simulink model "sim_dist_pos_obs_paper"  (R2020a)
settings: Solver=ode4  StartTime=0.0  StopTime=30.0  FixedStep=0.01  RelTol=1e-3
values from neighbouring files (symbols this model uses):
  alfa_theta = 20    [draw_compare_dist_pos_obs.m]
  alfa_theta_obs = 100    [draw_compare_dist_pos_obs.m]
  beta1 = 1.2    [draw_compare_dist_pos_obs.m]
  beta2 = 0.8    [draw_compare_dist_pos_obs.m]
  c1_diff_sigma_bar_v = diag([25; 30; 20])    [draw_compare_dist_pos_obs.m]
  c1v = diag([16.0; 16.0; 16.0])    [draw_compare_dist_pos_obs.m]
  c2_diff_sigma_bar_v = diag([50; 50; 10])    [draw_compare_dist_pos_obs.m]
  c2v = diag([16.0; 16.0; 16.0])    [draw_compare_dist_pos_obs.m]
  c3_diff_sigma_bar_v = diag([15; 15; 10])    [draw_compare_dist_pos_obs.m]
  c3v = diag([16.0; 16.0; 16.0])    [draw_compare_dist_pos_obs.m]
  delta_p_i_0 = zeros(3, NF)    [draw_compare_dist_pos_obs.m]
  delta_v_i_0 = zeros(3, NF)    [draw_compare_dist_pos_obs.m]
  dp_aa_t = 0.2 * ones(3, 5) + ( 1.0 - 0.2 ) * rand(3, 5)    [draw_compare_dist_pos_obs.m]
  dp_ff_t = [ 0.4 * ones(1, 5) + ( 1.0 - 0.4 ) * rand(1, 5);                      0.4 * ones(1, 5) + ( 1.0 - 0.4 ) * rand(1, 5);                      0.2 * ones(1, 5) + ( 0.6 - 0.2 ) * rand(1, 5) ]    [draw_compare_dist_pos_obs.m]
  dp_phi_t = ( - pi / 2 ) * ones(3, 5) + ( pi / 2 - ( - pi / 2 ) ) * rand(3, 5)    [draw_compare_dist_pos_obs.m]
  etai_0 = zeros(3,5)    [draw_compare_dist_pos_obs.m]
  kai_1_t = 0.02    [draw_compare_dist_pos_obs.m]
  kai_3_t = 0.1    [draw_compare_dist_pos_obs.m]
  kai_chi_1 = diag([6; 6; 6])    [draw_compare_dist_pos_obs.m]
  kai_chi_2 = diag([6; 6; 6])    [draw_compare_dist_pos_obs.m]
  kai_u_1 = diag([8; 8; 8])    [draw_compare_dist_pos_obs.m]
  kai_u_2 = diag([8; 8; 8])    [draw_compare_dist_pos_obs.m]
  ksii_0 = zeros(3,5)    [draw_compare_dist_pos_obs.m]
  l1v = diag([20; 20; 20])    [draw_compare_dist_pos_obs.m]
  l2v = diag([30; 30; 30])    [draw_compare_dist_pos_obs.m]
  Lamd_diff_sigma_bar_v = 0.5    [draw_compare_dist_pos_obs.m]
  mass_i = zeros(1,NF)    [draw_compare_dist_pos_obs.m]
  Mii = diag([1;0;0;0;1])    [draw_compare_dist_pos_obs.m]
  pos0 = zeros(3, 1)    [draw_compare_dist_pos_obs.m]
  PZ0 = P0(3)    [draw_compare_dist_pos_obs.m]
  PZ1 = 10    [draw_compare_dist_pos_obs.m]
  Qci_init = repmat([1;0;0;0],1,NF)    [draw_compare_dist_pos_obs.m]
  R0 = 4    [draw_compare_dist_pos_obs.m]
  R1 = 8    [draw_compare_dist_pos_obs.m]
  Rx2 = 10    [draw_compare_dist_pos_obs.m]
  Ry2 = 6    [draw_compare_dist_pos_obs.m]
  Rz2 = 4    [draw_compare_dist_pos_obs.m]
  T0 = 0    [draw_compare_dist_pos_obs.m]
  T1 = tseq1    (= 10)    [draw_compare_dist_pos_obs.m]
  T12 = tseq1 + tseq12    (= 20)    [draw_compare_dist_pos_obs.m]
  T2 = tseq1 + tseq12 + tseq2    (= 30)    [draw_compare_dist_pos_obs.m]
  theta0 = ( 2 / 5 ) * pi    (= 1.25663706144)    [draw_compare_dist_pos_obs.m]
  vel0 = zeros(3, 1)    [draw_compare_dist_pos_obs.m]
  Wij = [0,0,1,0,0;              0,0,1,1,0;              1,0,0,0,1;              0,1,1,0,0;              0,0,1,0,0]    [draw_compare_dist_pos_obs.m]
  X1 = 8    [draw_compare_dist_pos_obs.m]
  X2 = 2    [draw_compare_dist_pos_obs.m]
  X3 = 3    [draw_compare_dist_pos_obs.m]
  Y1 = 10    [draw_compare_dist_pos_obs.m]
  Y2 = 2    [draw_compare_dist_pos_obs.m]
  Y3 = 4    [draw_compare_dist_pos_obs.m]
  Z1 = 4    [draw_compare_dist_pos_obs.m]
  Z2 = -6    [draw_compare_dist_pos_obs.m]
  Z3 = 2    [draw_compare_dist_pos_obs.m]
  zeta_diff_sigma_bar_v = 0.08    [draw_compare_dist_pos_obs.m]
undefined symbols (not defined in the file or in its folder): cal_frac_squ, p_alfav1, p_alfav2, p_beta1, p_beta2, p_dbeta1, p_dbeta2, p_gamma1_pos, p_gamma1_vel, p_gamma2_pos, p_gamma2_vel, q_alfav1, q_alfav2, q_beta1, q_beta2, q_dbeta1, q_dbeta2, q_gamma1_pos, q_gamma1_vel, q_gamma2_pos, q_gamma2_vel
(part 1 of 5)
settings Model: Creator=zzy  LastModifiedBy=Hershey.A
settings DataIOCC: ReturnWorkspaceOutputs=off
settings DebuggingCC: ArithmeticOperatorsInVariantConditions=warning
settings SFSimCC: SimUseLocalCustomCode=off  CustomCodeUndefinedFunction=UseInterfaceOnly
settings RTWCC: RTWUseLocalCustomCode=off

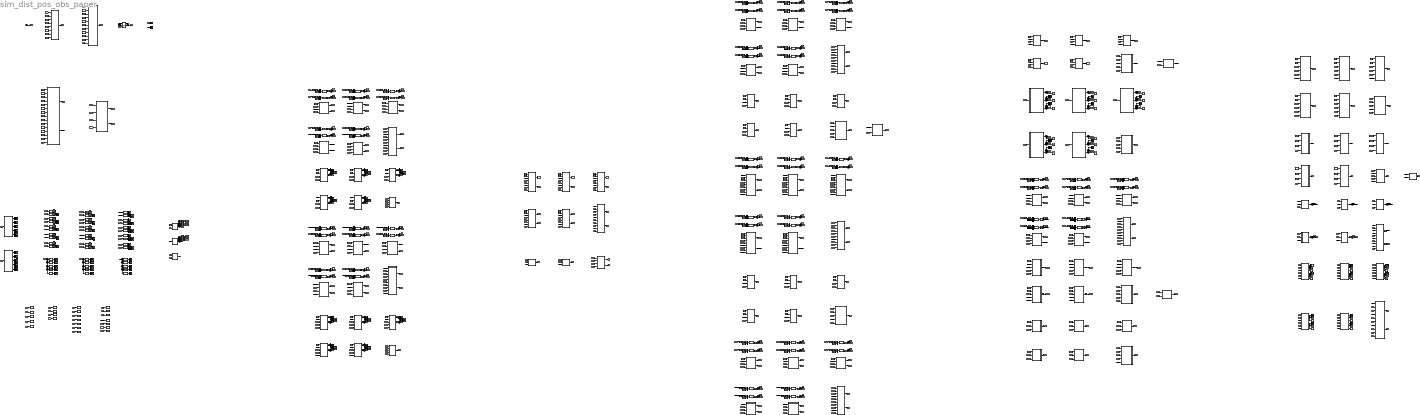
== system sim_dist_pos_obs_paper ==
  Add{,1..9} (10 alike) : Sum
  Clock : Clock
  Constant : Constant  Value=T1
  Constant{1,4,9,19,24,149,154,159,164,169} (10 alike) : Constant  Value=q_beta1
  Constant{5,10,14,16,20,39,46,54,61,79,101,103,108,113,118,148,153,158,163,168} (20 alike) : Constant  Value=alfa_theta
  Constant{100,102,107,112,117} (5 alike) : Constant  Value=p_alfav1
  Constant{97,104,109,114,119} (5 alike) : Constant  Value=q_alfav1
  Constant{98,105,110,115,120} (5 alike) : Constant  Value=p_alfav2
  Constant{99,106,111,116,121} (5 alike) : Constant  Value=q_alfav2
  Constant{2,6,11,15,21,150,155,160,165,170} (10 alike) : Constant  Value=p_beta2
  Constant{3,7,12,17,22,151,156,161,166,171} (10 alike) : Constant  Value=q_beta2
  Constant{122,124,126,128,140} (5 alike) : Constant  Value=c1v
  Constant{123,125,127,139,141} (5 alike) : Constant  Value=c2v
  Constant129 : Constant  Value=R0
  Constant{8,13,18,23,63,147,152,157,162,167} (10 alike) : Constant  Value=p_beta1
  Constant130 : Constant  Value=R1
  Constant131 : Constant  Value=T0
  Constant132 : Constant  Value=Rz2
  Constant133 : Constant  Value=Ry2
  Constant134 : Constant  Value=Rx2
  Constant135 : Constant  Value=X1
  Constant136 : Constant  Value=X2
  Constant137 : Constant  Value=Y1
  Constant138 : Constant  Value=Y2
  Constant{92..96,142..146} (10 alike) : Constant  Value=c3v
  Constant{172,174,176,178,180} (5 alike) : Constant  Value=kai_u_1
  Constant{173,175,177,179,181} (5 alike) : Constant  Value=kai_u_2
  Constant{182..183,189,199,202,205,209,212,219,252} (10 alike) : Constant  Value=l2v
  Constant{184..186,193..196,198,283..284} (10 alike) : Constant  Value=alfa_theta_obs
  Constant{187,190,197,200,203,206,210,213,230,263} (10 alike) : Constant  Value=l1v
  Constant188 : Constant  Value=delta_p_i_0(:,4)
  Constant191 : Constant  Value=mass_i
  Constant192 : Constant  Value=delta_p_i_0(:,5)
  Constant201 : Constant  Value=delta_v_i_0(:,1)
  Constant204 : Constant  Value=delta_v_i_0(:,2)
  Constant207 : Constant  Value=delta_v_i_0(:,3)
  Constant208 : Constant  Value=delta_p_i_0(:,1)
  Constant211 : Constant  Value=delta_v_i_0(:,4)
  Constant214 : Constant  Value=delta_v_i_0(:,5)
  Constant{215,220,270,275,279} (5 alike) : Constant  Value=p_gamma1_pos
  Constant{216,267,271,276,280} (5 alike) : Constant  Value=q_gamma1_pos
  Constant{217,268,272,277,281} (5 alike) : Constant  Value=p_gamma2_pos
  Constant{218,269,273,278,282} (5 alike) : Constant  Value=q_gamma2_pos
  Constant221 : Constant  Value=Z1
  Constant222 : Constant  Value=Z2
  Constant{223,227,232,236,240} (5 alike) : Constant  Value=Wij
  Constant{224,228,233,237,242} (5 alike) : Constant  Value=Mii
  Constant225 : Constant  Value=theta0
  Constant226 : Constant  Value=Z3
  Constant229 : Constant  Value=Y3
  Constant231 : Constant  Value=kai_1_t
  Constant234 : Constant  Value=X3
  Constant235 : Constant  Value=kai_3_t
  Constant238 : Constant  Value=T1
  Constant239 : Constant  Value=T12
  Constant241 : Constant  Value=delta_p_i_0(:,2)
  Constant{243,286,289,292,295} (5 alike) : Constant  Value=dp_phi_t
  Constant{244,287,290,293,296} (5 alike) : Constant  Value=dp_ff_t
  Constant{245,249,254,258,262} (5 alike) : Constant  Value=p_gamma1_vel
  Constant{246,250,255,259,264} (5 alike) : Constant  Value=q_gamma1_vel
  Constant{247,251,256,260,265} (5 alike) : Constant  Value=p_gamma2_vel
  Constant{248,253,257,261,266} (5 alike) : Constant  Value=q_gamma2_vel
  Constant{25,27,29,31,33,82,84,86,88,90} (10 alike) : Constant  Value=kai_chi_2
  Constant{26,28,30,32,34,83,85,87,89,91} (10 alike) : Constant  Value=kai_chi_1
  Constant274 : Constant  Value=delta_p_i_0(:,3)
  Constant{285,288,291,294,297} (5 alike) : Constant  Value=dp_aa_t
  Constant{35,42,49,57,75} (5 alike) : Constant  Value=q_dbeta1
  Constant{36,43,50,58,76} (5 alike) : Constant  Value=p_dbeta2
  Constant{37,44,52,59,77} (5 alike) : Constant  Value=q_dbeta2
  Constant{38,45,53,60,78} (5 alike) : Constant  Value=p_dbeta1
  Constant{40,47,55,62,80} (5 alike) : Constant  Value=beta1
  Constant{41,48,56,74,81} (5 alike) : Constant  Value=beta2
  Constant51 : Constant  Value=Qci_init
  Constant64 : Constant  Value=T2
  Constant65 : Constant  Value=R0
  Constant66 : Constant  Value=R1
  Constant67 : Constant  Value=Rx2
  Constant68 : Constant  Value=Ry2
  Constant69 : Constant  Value=Rz2
  Constant70 : Constant  Value=T2
  Constant71 : Constant  Value=T1
  Constant72 : Constant  Value=PZ0
  Constant73 : Constant  Value=PZ1
  Demux{1..97} (97 alike) : Demux  Outputs=3
  Display{1..95} (95 alike) : Display
  Interpreted MATLAB Function{1..60} (60 alike) : MATLABFcn  MATLABFcn=cal_frac_squ(u(1:3),u(4),u(5))
  Memory1 : Memory  InitialCondition=etai_0
  Memory2 : Memory  InitialCondition=ksii_0
  Mux{1..40,109..118,120..129} (60 alike) : Mux  Inputs=3
  Mux{41..108,119,130..135} (75 alike) : Mux  Inputs=2
  Step : Step  Time=T1+0.01  SampleTime=0
  To Workspace : ToWorkspace  VariableName=eta_d_est_vec  SampleTime=-1
  To Workspace1 : ToWorkspace  VariableName=dp_hat_vec  SampleTime=-1
  To Workspace10 : ToWorkspace  VariableName=eta_track_err_vec  SampleTime=-1
  To Workspace11 : ToWorkspace  VariableName=sigma_bar_v_hat_vec  SampleTime=-1
  To Workspace12 : ToWorkspace  VariableName=sigma_bar_v_vec  SampleTime=-1
  To Workspace13 : ToWorkspace  VariableName=sigma_bar_v_tilt_vec  SampleTime=-1
  To Workspace14 : ToWorkspace  VariableName=ui_vec  SampleTime=-1
  To Workspace15 : ToWorkspace  VariableName=chi_vec  SampleTime=-1
  To Workspace16 : ToWorkspace  VariableName=phi_vec  SampleTime=-1
  To Workspace17 : ToWorkspace  VariableName=ksi_est_err  SampleTime=-1
  To Workspace18 : ToWorkspace  VariableName=ksi_d_est_vec  SampleTime=-1
  To Workspace19 : ToWorkspace  VariableName=sigma_v_vec  SampleTime=-1
  To Workspace2 : ToWorkspace  VariableName=dp_vec  SampleTime=-1
  To Workspace20 : ToWorkspace  VariableName=delta_ksi_vec  SampleTime=-1
  To Workspace21 : ToWorkspace  VariableName=delta_eta_vec  SampleTime=-1
  To Workspace22 : ToWorkspace  VariableName=eta_est_err  SampleTime=-1
  To Workspace3 : ToWorkspace  VariableName=u0  SampleTime=-1
  To Workspace4 : ToWorkspace  VariableName=eta0  SampleTime=-1
  To Workspace5 : ToWorkspace  VariableName=ksi0  SampleTime=-1
  To Workspace6 : ToWorkspace  VariableName=dp_tilt_vec  SampleTime=-1
  To Workspace7 : ToWorkspace  VariableName=eta_i_vec  SampleTime=-1
  To Workspace8 : ToWorkspace  VariableName=ksi_i_vec  SampleTime=-1
  To Workspace9 : ToWorkspace  VariableName=ksi_track_err_vec  SampleTime=-1
  cal Rci from ui : MATLAB Function  TreatAsAtomicUnit=on
  cal Rei : MATLAB Function  TreatAsAtomicUnit=on
  cal Ri : MATLAB Function  TreatAsAtomicUnit=on
  cal abs 1 : MATLAB Function  TreatAsAtomicUnit=on
  cal abs 10 : MATLAB Function  TreatAsAtomicUnit=on
  cal abs 11 : MATLAB Function  TreatAsAtomicUnit=on
  cal abs 12 : MATLAB Function  TreatAsAtomicUnit=on
  cal abs 13 : MATLAB Function  TreatAsAtomicUnit=on
  cal abs 14 : MATLAB Function  TreatAsAtomicUnit=on
  cal abs 15 : MATLAB Function  TreatAsAtomicUnit=on
  cal abs 16 : MATLAB Function  TreatAsAtomicUnit=on
  cal abs 17 : MATLAB Function  TreatAsAtomicUnit=on
  cal abs 18 : MATLAB Function  TreatAsAtomicUnit=on
  cal abs 19 : MATLAB Function  TreatAsAtomicUnit=on
  cal abs 2 : MATLAB Function  TreatAsAtomicUnit=on
  cal abs 20 : MATLAB Function  TreatAsAtomicUnit=on
  cal abs 21 : MATLAB Function  TreatAsAtomicUnit=on
  cal abs 22 : MATLAB Function  TreatAsAtomicUnit=on
  cal abs 23 : MATLAB Function  TreatAsAtomicUnit=on
  cal abs 24 : MATLAB Function  TreatAsAtomicUnit=on
  cal abs 25 : MATLAB Function  TreatAsAtomicUnit=on
  cal abs 26 : MATLAB Function  TreatAsAtomicUnit=on
  cal abs 27 : MATLAB Function  TreatAsAtomicUnit=on
  cal abs 28 : MATLAB Function  TreatAsAtomicUnit=on
  cal abs 29 : MATLAB Function  TreatAsAtomicUnit=on
  cal abs 3 : MATLAB Function  TreatAsAtomicUnit=on
  cal abs 30 : MATLAB Function  TreatAsAtomicUnit=on
  cal abs 31 : MATLAB Function  TreatAsAtomicUnit=on
  cal abs 32 : MATLAB Function  TreatAsAtomicUnit=on
  cal abs 33 : MATLAB Function  TreatAsAtomicUnit=on
  cal abs 34 : MATLAB Function  TreatAsAtomicUnit=on
  cal abs 35 : MATLAB Function  TreatAsAtomicUnit=on
  cal abs 36 : MATLAB Function  TreatAsAtomicUnit=on
  cal abs 37 : MATLAB Function  TreatAsAtomicUnit=on
  cal abs 38 : MATLAB Function  TreatAsAtomicUnit=on
  cal abs 39 : MATLAB Function  TreatAsAtomicUnit=on
  cal abs 4 : MATLAB Function  TreatAsAtomicUnit=on
  cal abs 40 : MATLAB Function  TreatAsAtomicUnit=on
  cal abs 41 : MATLAB Function  TreatAsAtomicUnit=on
  cal abs 42 : MATLAB Function  TreatAsAtomicUnit=on
  cal abs 43 : MATLAB Function  TreatAsAtomicUnit=on
  cal abs 44 : MATLAB Function  TreatAsAtomicUnit=on
  cal abs 45 : MATLAB Function  TreatAsAtomicUnit=on
  cal abs 46 : MATLAB Function  TreatAsAtomicUnit=on
  cal abs 47 : MATLAB Function  TreatAsAtomicUnit=on
  cal abs 48 : MATLAB Function  TreatAsAtomicUnit=on
  cal abs 49 : MATLAB Function  TreatAsAtomicUnit=on
  cal abs 5 : MATLAB Function  TreatAsAtomicUnit=on
  cal abs 50 : MATLAB Function  TreatAsAtomicUnit=on
  cal abs 51 : MATLAB Function  TreatAsAtomicUnit=on
  cal abs 52 : MATLAB Function  TreatAsAtomicUnit=on
  cal abs 53 : MATLAB Function  TreatAsAtomicUnit=on
  cal abs 54 : MATLAB Function  TreatAsAtomicUnit=on
  cal abs 55 : MATLAB Function  TreatAsAtomicUnit=on
  cal abs 56 : MATLAB Function  TreatAsAtomicUnit=on
  cal abs 57 : MATLAB Function  TreatAsAtomicUnit=on
  cal abs 58 : MATLAB Function  TreatAsAtomicUnit=on
  cal abs 59 : MATLAB Function  TreatAsAtomicUnit=on
  cal abs 6 : MATLAB Function  TreatAsAtomicUnit=on
  cal abs 60 : MATLAB Function  TreatAsAtomicUnit=on
  cal abs 7 : MATLAB Function  TreatAsAtomicUnit=on
  cal abs 8 : MATLAB Function  TreatAsAtomicUnit=on
  cal abs 9 : MATLAB Function  TreatAsAtomicUnit=on
  cal combine sigma_bar_v : MATLAB Function  TreatAsAtomicUnit=on
  cal combine sigma_bar_v_tilt : MATLAB Function  TreatAsAtomicUnit=on
  cal d_theta_err_ksi agent 1 : MATLAB Function  TreatAsAtomicUnit=on
  cal d_theta_err_ksi agent 2 : MATLAB Function  TreatAsAtomicUnit=on
  cal d_theta_err_ksi agent 3 : MATLAB Function  TreatAsAtomicUnit=on
  cal d_theta_err_ksi agent 4 : MATLAB Function  TreatAsAtomicUnit=on
  cal d_theta_err_ksi agent 5 : MATLAB Function  TreatAsAtomicUnit=on
  cal dchi agent 1 : MATLAB Function  TreatAsAtomicUnit=on
  cal dchi agent 2 : MATLAB Function  TreatAsAtomicUnit=on
  cal dchi agent 3 : MATLAB Function  TreatAsAtomicUnit=on
  cal dchi agent 4 : MATLAB Function  TreatAsAtomicUnit=on
  cal dchi agent 5 : MATLAB Function  TreatAsAtomicUnit=on
  cal differentiator d_sigma_bar_v_hat agent 1 : Subsystem
  cal differentiator d_sigma_bar_v_hat agent 2 : Subsystem
  cal differentiator d_sigma_bar_v_hat agent 3 : Subsystem
  cal differentiator d_sigma_bar_v_hat agent 4 : Subsystem
  cal differentiator d_sigma_bar_v_hat agent 5 : Subsystem
  cal disturbance observation error dp_tilt : MATLAB Function  TreatAsAtomicUnit=on
  cal dp_hat agent 1 : MATLAB Function  TreatAsAtomicUnit=on
  cal dp_hat agent 2 : MATLAB Function  TreatAsAtomicUnit=on
  cal dp_hat agent 3 : MATLAB Function  TreatAsAtomicUnit=on
  cal dp_hat agent 4 : MATLAB Function  TreatAsAtomicUnit=on
  cal dp_hat agent 5 : MATLAB Function  TreatAsAtomicUnit=on
  cal formation tracking position and velocity errors : MATLAB Function  TreatAsAtomicUnit=on
  cal lumped observation error agent 1 : MATLAB Function  TreatAsAtomicUnit=on
  cal lumped observation error agent 2 : MATLAB Function  TreatAsAtomicUnit=on
  cal lumped observation error agent 3 : MATLAB Function  TreatAsAtomicUnit=on
  cal lumped observation error agent 4 : MATLAB Function  TreatAsAtomicUnit=on
  cal lumped observation error agent 5 : MATLAB Function  TreatAsAtomicUnit=on
  cal position estimate error : MATLAB Function  TreatAsAtomicUnit=on
  cal sigma_bar_v_hat agent 1 : MATLAB Function  TreatAsAtomicUnit=on
  cal sigma_bar_v_hat agent 2 : MATLAB Function  TreatAsAtomicUnit=on
  cal sigma_bar_v_hat agent 3 : MATLAB Function  TreatAsAtomicUnit=on
  cal sigma_bar_v_hat agent 4 : MATLAB Function  TreatAsAtomicUnit=on
  cal sigma_bar_v_hat agent 5 : MATLAB Function  TreatAsAtomicUnit=on
  cal theta_err_ksi agent 1 : MATLAB Function  TreatAsAtomicUnit=on
  cal theta_err_ksi agent 2 : MATLAB Function  TreatAsAtomicUnit=on
  cal theta_err_ksi agent 3 : MATLAB Function  TreatAsAtomicUnit=on
  cal theta_err_ksi agent 4 : MATLAB Function  TreatAsAtomicUnit=on
  cal theta_err_ksi agent 5 : MATLAB Function  TreatAsAtomicUnit=on
  cal theta_eta_est_err_tilt agent 1 : MATLAB Function  TreatAsAtomicUnit=on
  cal theta_eta_est_err_tilt agent 2 : MATLAB Function  TreatAsAtomicUnit=on
  cal theta_eta_est_err_tilt agent 3 : MATLAB Function  TreatAsAtomicUnit=on
  cal theta_eta_est_err_tilt agent 4 : MATLAB Function  TreatAsAtomicUnit=on
  cal theta_eta_est_err_tilt agent 5 : MATLAB Function  TreatAsAtomicUnit=on
  cal theta_ksi_est_err_tilt agent 1 : MATLAB Function  TreatAsAtomicUnit=on
  cal theta_ksi_est_err_tilt agent 2 : MATLAB Function  TreatAsAtomicUnit=on
  cal theta_ksi_est_err_tilt agent 3 : MATLAB Function  TreatAsAtomicUnit=on
  cal theta_ksi_est_err_tilt agent 4 : MATLAB Function  TreatAsAtomicUnit=on
  cal theta_ksi_est_err_tilt agent 5 : MATLAB Function  TreatAsAtomicUnit=on
  cal theta_phi agent 1 : MATLAB Function  TreatAsAtomicUnit=on
  cal theta_phi agent 2 : MATLAB Function  TreatAsAtomicUnit=on
  cal theta_phi agent 3 : MATLAB Function  TreatAsAtomicUnit=on
  cal theta_phi agent 4 : MATLAB Function  TreatAsAtomicUnit=on
  cal theta_phi agent 5 : MATLAB Function  TreatAsAtomicUnit=on
  cal theta_sigma_bar_v_tilt agent 1 : MATLAB Function  TreatAsAtomicUnit=on
  cal theta_sigma_bar_v_tilt agent 2 : MATLAB Function  TreatAsAtomicUnit=on
  cal theta_sigma_bar_v_tilt agent 3 : MATLAB Function  TreatAsAtomicUnit=on
  cal theta_sigma_bar_v_tilt agent 4 : MATLAB Function  TreatAsAtomicUnit=on
  cal theta_sigma_bar_v_tilt agent 5 : MATLAB Function  TreatAsAtomicUnit=on
  cal ui agent 1 : MATLAB Function  TreatAsAtomicUnit=on
  cal ui agent 2 : MATLAB Function  TreatAsAtomicUnit=on
  cal ui agent 3 : MATLAB Function  TreatAsAtomicUnit=on
  cal ui agent 4 : MATLAB Function  TreatAsAtomicUnit=on
  cal ui agent 5 : MATLAB Function  TreatAsAtomicUnit=on
  cal velocity estimate error : MATLAB Function  TreatAsAtomicUnit=on
  cal virtual control sigma_v agent 1 : MATLAB Function  TreatAsAtomicUnit=on
  cal virtual control sigma_v agent 2 : MATLAB Function  TreatAsAtomicUnit=on
  cal virtual control sigma_v agent 3 : MATLAB Function  TreatAsAtomicUnit=on
  cal virtual control sigma_v agent 4 : MATLAB Function  TreatAsAtomicUnit=on
  cal virtual control sigma_v agent 5 : MATLAB Function  TreatAsAtomicUnit=on
  cal virtual velocity control error phi : MATLAB Function  TreatAsAtomicUnit=on
  choose chi_1 : MATLAB Function  TreatAsAtomicUnit=on
  choose chi_2 : MATLAB Function  TreatAsAtomicUnit=on
  choose chi_3 : MATLAB Function  TreatAsAtomicUnit=on
  choose chi_4 : MATLAB Function  TreatAsAtomicUnit=on
  choose chi_5 : MATLAB Function  TreatAsAtomicUnit=on
  choose dp_1 : MATLAB Function  TreatAsAtomicUnit=on
  choose dp_2 : MATLAB Function  TreatAsAtomicUnit=on
  choose dp_3 : MATLAB Function  TreatAsAtomicUnit=on
  choose dp_4 : MATLAB Function  TreatAsAtomicUnit=on
  choose dp_5 : MATLAB Function  TreatAsAtomicUnit=on
  choose dp_hat_1 : MATLAB Function  TreatAsAtomicUnit=on
  choose dp_hat_2 : MATLAB Function  TreatAsAtomicUnit=on
  choose dp_hat_3 : MATLAB Function  TreatAsAtomicUnit=on
  choose dp_hat_4 : MATLAB Function  TreatAsAtomicUnit=on
  choose dp_hat_5 : MATLAB Function  TreatAsAtomicUnit=on
  choose dp_tilt_1 : MATLAB Function  TreatAsAtomicUnit=on
  choose dp_tilt_2 : MATLAB Function  TreatAsAtomicUnit=on
  choose dp_tilt_3 : MATLAB Function  TreatAsAtomicUnit=on
  choose dp_tilt_4 : MATLAB Function  TreatAsAtomicUnit=on
  choose dp_tilt_5 : MATLAB Function  TreatAsAtomicUnit=on
  choose err_eta_1 : MATLAB Function  TreatAsAtomicUnit=on
  choose err_eta_2 : MATLAB Function  TreatAsAtomicUnit=on
  choose err_eta_3 : MATLAB Function  TreatAsAtomicUnit=on
  choose err_eta_4 : MATLAB Function  TreatAsAtomicUnit=on
  choose err_eta_5 : MATLAB Function  TreatAsAtomicUnit=on
  choose eta_est_err_tilt 1 : MATLAB Function  TreatAsAtomicUnit=on
  choose eta_est_err_tilt 10 : MATLAB Function  TreatAsAtomicUnit=on
  choose eta_est_err_tilt 11 : MATLAB Function  TreatAsAtomicUnit=on
  choose eta_est_err_tilt 12 : MATLAB Function  TreatAsAtomicUnit=on
  choose eta_est_err_tilt 13 : MATLAB Function  TreatAsAtomicUnit=on
  choose eta_est_err_tilt 14 : MATLAB Function  TreatAsAtomicUnit=on
  choose eta_est_err_tilt 15 : MATLAB Function  TreatAsAtomicUnit=on
  choose eta_est_err_tilt 16 : MATLAB Function  TreatAsAtomicUnit=on
  choose eta_est_err_tilt 17 : MATLAB Function  TreatAsAtomicUnit=on
  choose eta_est_err_tilt 18 : MATLAB Function  TreatAsAtomicUnit=on
  choose eta_est_err_tilt 19 : MATLAB Function  TreatAsAtomicUnit=on
  choose eta_est_err_tilt 2 : MATLAB Function  TreatAsAtomicUnit=on
  choose eta_est_err_tilt 20 : MATLAB Function  TreatAsAtomicUnit=on
  choose eta_est_err_tilt 3 : MATLAB Function  TreatAsAtomicUnit=on
  choose eta_est_err_tilt 4 : MATLAB Function  TreatAsAtomicUnit=on
  choose eta_est_err_tilt 5 : MATLAB Function  TreatAsAtomicUnit=on
  choose eta_est_err_tilt 6 : MATLAB Function  TreatAsAtomicUnit=on
  choose eta_est_err_tilt 7 : MATLAB Function  TreatAsAtomicUnit=on
  choose eta_est_err_tilt 8 : MATLAB Function  TreatAsAtomicUnit=on
  choose eta_est_err_tilt 9 : MATLAB Function  TreatAsAtomicUnit=on
  choose ksi_est_err 1 : MATLAB Function  TreatAsAtomicUnit=on
  choose ksi_est_err 10 : MATLAB Function  TreatAsAtomicUnit=on
  choose ksi_est_err 11 : MATLAB Function  TreatAsAtomicUnit=on
  choose ksi_est_err 12 : MATLAB Function  TreatAsAtomicUnit=on
  choose ksi_est_err 13 : MATLAB Function  TreatAsAtomicUnit=on
  choose ksi_est_err 14 : MATLAB Function  TreatAsAtomicUnit=on
  choose ksi_est_err 15 : MATLAB Function  TreatAsAtomicUnit=on
  choose ksi_est_err 16 : MATLAB Function  TreatAsAtomicUnit=on
  choose ksi_est_err 17 : MATLAB Function  TreatAsAtomicUnit=on
  choose ksi_est_err 18 : MATLAB Function  TreatAsAtomicUnit=on
  choose ksi_est_err 19 : MATLAB Function  TreatAsAtomicUnit=on
  choose ksi_est_err 2 : MATLAB Function  TreatAsAtomicUnit=on
  choose ksi_est_err 20 : MATLAB Function  TreatAsAtomicUnit=on
  choose ksi_est_err 21 : MATLAB Function  TreatAsAtomicUnit=on
  choose ksi_est_err 22 : MATLAB Function  TreatAsAtomicUnit=on
  choose ksi_est_err 23 : MATLAB Function  TreatAsAtomicUnit=on
  choose ksi_est_err 24 : MATLAB Function  TreatAsAtomicUnit=on
  choose ksi_est_err 25 : MATLAB Function  TreatAsAtomicUnit=on
  choose ksi_est_err 26 : MATLAB Function  TreatAsAtomicUnit=on
  choose ksi_est_err 27 : MATLAB Function  TreatAsAtomicUnit=on
  choose ksi_est_err 28 : MATLAB Function  TreatAsAtomicUnit=on
  choose ksi_est_err 29 : MATLAB Function  TreatAsAtomicUnit=on
  choose ksi_est_err 3 : MATLAB Function  TreatAsAtomicUnit=on
  choose ksi_est_err 30 : MATLAB Function  TreatAsAtomicUnit=on
  choose ksi_est_err 31 : MATLAB Function  TreatAsAtomicUnit=on
  choose ksi_est_err 32 : MATLAB Function  TreatAsAtomicUnit=on
  choose ksi_est_err 33 : MATLAB Function  TreatAsAtomicUnit=on
  choose ksi_est_err 34 : MATLAB Function  TreatAsAtomicUnit=on
  choose ksi_est_err 35 : MATLAB Function  TreatAsAtomicUnit=on
  choose ksi_est_err 36 : MATLAB Function  TreatAsAtomicUnit=on
  choose ksi_est_err 37 : MATLAB Function  TreatAsAtomicUnit=on
  choose ksi_est_err 38 : MATLAB Function  TreatAsAtomicUnit=on
  choose ksi_est_err 39 : MATLAB Function  TreatAsAtomicUnit=on
  choose ksi_est_err 4 : MATLAB Function  TreatAsAtomicUnit=on
  choose ksi_est_err 40 : MATLAB Function  TreatAsAtomicUnit=on
  choose ksi_est_err 5 : MATLAB Function  TreatAsAtomicUnit=on
  choose ksi_est_err 6 : MATLAB Function  TreatAsAtomicUnit=on
  choose ksi_est_err 7 : MATLAB Function  TreatAsAtomicUnit=on
  choose ksi_est_err 8 : MATLAB Function  TreatAsAtomicUnit=on
  choose ksi_est_err 9 : MATLAB Function  TreatAsAtomicUnit=on
  choose phi_1 : MATLAB Function  TreatAsAtomicUnit=on
  choose phi_2 : MATLAB Function  TreatAsAtomicUnit=on
  choose phi_3 : MATLAB Function  TreatAsAtomicUnit=on
  choose phi_4 : MATLAB Function  TreatAsAtomicUnit=on
  choose phi_5 : MATLAB Function  TreatAsAtomicUnit=on
  choose sigma_bar_v_1 : MATLAB Function  TreatAsAtomicUnit=on
  choose sigma_bar_v_2 : MATLAB Function  TreatAsAtomicUnit=on
  choose sigma_bar_v_3 : MATLAB Function  TreatAsAtomicUnit=on
  choose sigma_bar_v_4 : MATLAB Function  TreatAsAtomicUnit=on
  choose sigma_bar_v_5 : MATLAB Function  TreatAsAtomicUnit=on
  choose sigma_bar_v_hat_1 : MATLAB Function  TreatAsAtomicUnit=on
  choose sigma_bar_v_hat_2 : MATLAB Function  TreatAsAtomicUnit=on
  choose sigma_bar_v_hat_3 : MATLAB Function  TreatAsAtomicUnit=on
  choose sigma_bar_v_hat_4 : MATLAB Function  TreatAsAtomicUnit=on
  choose sigma_bar_v_hat_5 : MATLAB Function  TreatAsAtomicUnit=on
  choose sigma_bar_v_tilt_1 : MATLAB Function  TreatAsAtomicUnit=on
  choose sigma_bar_v_tilt_2 : MATLAB Function  TreatAsAtomicUnit=on
  choose sigma_bar_v_tilt_3 : MATLAB Function  TreatAsAtomicUnit=on
  choose sigma_bar_v_tilt_4 : MATLAB Function  TreatAsAtomicUnit=on
  choose sigma_bar_v_tilt_5 : MATLAB Function  TreatAsAtomicUnit=on
  combine chi : MATLAB Function  TreatAsAtomicUnit=on
  combine d_sigma_bar_v_est : MATLAB Function  TreatAsAtomicUnit=on
  combine dchi : MATLAB Function  TreatAsAtomicUnit=on
  combine dp_hat : MATLAB Function  TreatAsAtomicUnit=on
  combine dtheta_err_ksi : MATLAB Function  TreatAsAtomicUnit=on
  combine follower desire velocity estimaters : MATLAB Function  TreatAsAtomicUnit=on
  combine follower eta ksi : MATLAB Function  TreatAsAtomicUnit=on
  combine formation control input : MATLAB Function  TreatAsAtomicUnit=on
  combine leader position estimaters : MATLAB Function  TreatAsAtomicUnit=on
  "combine lumped follower observation error " : MATLAB Function  TreatAsAtomicUnit=on
  combine lumped follower position observation error : MATLAB Function  TreatAsAtomicUnit=on
  combine lumped follower velocity observation error : MATLAB Function  TreatAsAtomicUnit=on
  combine sigma_bar_v_hat : MATLAB Function  TreatAsAtomicUnit=on
  combine sigma_v : MATLAB Function  TreatAsAtomicUnit=on
  combine theta_err_ksi : MATLAB Function  TreatAsAtomicUnit=on
  combine theta_err_ksi1 : MATLAB Function  TreatAsAtomicUnit=on
  combine theta_sigma_bar_v_tilt : MATLAB Function  TreatAsAtomicUnit=on
  combine translational disturbance : MATLAB Function  TreatAsAtomicUnit=on
  combine ui : MATLAB Function  TreatAsAtomicUnit=on
  compare dp_1 and dp_hat_1 : Scope  NumInputPorts=3
  compare dp_2 and dp_hat_2 : Scope  NumInputPorts=3
  compare dp_3 and dp_hat_3 : Scope  NumInputPorts=3
  compare dp_4 and dp_hat_4 : Scope  NumInputPorts=3
  compare dp_5 and dp_hat_5 : Scope  NumInputPorts=3
  compare err_eta_1 and chi_1 : Scope  NumInputPorts=3
  compare err_eta_2 and chi_2 : Scope  NumInputPorts=3
  compare err_eta_3 and chi_3 : Scope  NumInputPorts=3
  compare err_eta_4 and chi_4 : Scope  NumInputPorts=3
  compare err_eta_5 and chi_5 : Scope  NumInputPorts=3
  compare sigma_bar_v_1 and sigma_bar_v_hat_1 : Scope  NumInputPorts=3
  compare sigma_bar_v_2 and sigma_bar_v_hat_2 : Scope  NumInputPorts=3
  compare sigma_bar_v_3 and sigma_bar_v_hat_3 : Scope  NumInputPorts=3
  compare sigma_bar_v_4 and sigma_bar_v_hat_4 : Scope  NumInputPorts=3
  compare sigma_bar_v_5 and sigma_bar_v_hat_5 : Scope  NumInputPorts=3
  d2_sigma_bar_v_est_{1..5} (5 alike) : Scope  NumInputPorts=3
  d_sigma_bar_v_est_{1..5} (5 alike) : Scope  NumInputPorts=3
  depart Rc1 : MATLAB Function  TreatAsAtomicUnit=on
  depart Rc2 : MATLAB Function  TreatAsAtomicUnit=on
  depart Rc3 : MATLAB Function  TreatAsAtomicUnit=on
  depart Rc4 : MATLAB Function  TreatAsAtomicUnit=on
  depart Rc5 : MATLAB Function  TreatAsAtomicUnit=on
  depart Re1 : MATLAB Function  TreatAsAtomicUnit=on
  depart Re2 : MATLAB Function  TreatAsAtomicUnit=on
  depart Re3 : MATLAB Function  TreatAsAtomicUnit=on
  depart Re4 : MATLAB Function  TreatAsAtomicUnit=on
  depart Re5 : MATLAB Function  TreatAsAtomicUnit=on
  desire formation position and velocity : MATLAB Function  TreatAsAtomicUnit=on
  divide eta_est_err : MATLAB Function  TreatAsAtomicUnit=on
  divide ksi_est_err : MATLAB Function  TreatAsAtomicUnit=on
  dp_tilt_{1..5} (5 alike) : Scope  NumInputPorts=3
  eta_0 : Scope  NumInputPorts=3
  eta_d_est_{1..5} (5 alike) : Scope  NumInputPorts=3
  eta_est_err_{1..5} (5 alike) : Scope  NumInputPorts=3
  eta_track_err_{1..5} (5 alike) : Scope  NumInputPorts=3
  fixed-time distributed follower desire position observer agent 1 : MATLAB Function  TreatAsAtomicUnit=on
  fixed-time distributed follower desire position observer agent 2 : MATLAB Function  TreatAsAtomicUnit=on
  fixed-time distributed follower desire position observer agent 3 : MATLAB Function  TreatAsAtomicUnit=on
  fixed-time distributed follower desire position observer agent 4 : MATLAB Function  TreatAsAtomicUnit=on
  fixed-time distributed follower desire position observer agent 5 : MATLAB Function  TreatAsAtomicUnit=on
  fixed-time distributed follower desire velocity observer agent 1 : MATLAB Function  TreatAsAtomicUnit=on
  fixed-time distributed follower desire velocity observer agent 2 : MATLAB Function  TreatAsAtomicUnit=on
  fixed-time distributed follower desire velocity observer agent 3 : MATLAB Function  TreatAsAtomicUnit=on
  fixed-time distributed follower desire velocity observer agent 4 : MATLAB Function  TreatAsAtomicUnit=on
  fixed-time distributed follower desire velocity observer agent 5 : MATLAB Function  TreatAsAtomicUnit=on
  follower etai Integrator agent 1 : Integrator  InitialCondition=etai_0(:,1)
  follower etai Integrator agent 2 : Integrator  InitialCondition=etai_0(:,2)
  follower etai Integrator agent 3 : Integrator  InitialCondition=etai_0(:,3)
  follower etai Integrator agent 4 : Integrator  InitialCondition=etai_0(:,4)
  follower etai Integrator agent 5 : Integrator  InitialCondition=etai_0(:,5)
  follower ksii Integrator agent 1 : Integrator  InitialCondition=ksii_0(:,1)
  follower ksii Integrator agent 2 : Integrator  InitialCondition=ksii_0(:,2)
  follower ksii Integrator agent 3 : Integrator  InitialCondition=ksii_0(:,3)
  follower ksii Integrator agent 4 : Integrator  InitialCondition=ksii_0(:,4)
  follower ksii Integrator agent 5 : Integrator  InitialCondition=ksii_0(:,5)
  follower tracking error agent 1 : MATLAB Function  TreatAsAtomicUnit=on
  follower tracking error agent 2 : MATLAB Function  TreatAsAtomicUnit=on
  follower tracking error agent 3 : MATLAB Function  TreatAsAtomicUnit=on
  follower tracking error agent 4 : MATLAB Function  TreatAsAtomicUnit=on
  follower tracking error agent 5 : MATLAB Function  TreatAsAtomicUnit=on
  generate translational disturbance agent 1 : MATLAB Function  TreatAsAtomicUnit=on
  generate translational disturbance agent 2 : MATLAB Function  TreatAsAtomicUnit=on
  generate translational disturbance agent 3 : MATLAB Function  TreatAsAtomicUnit=on
  generate translational disturbance agent 4 : MATLAB Function  TreatAsAtomicUnit=on
  generate translational disturbance agent 5 : MATLAB Function  TreatAsAtomicUnit=on
  ksi_0 : Scope  NumInputPorts=3
  ksi_d_est_{1..5} (5 alike) : Scope  NumInputPorts=3
  ksi_est_err_{1..5} (5 alike) : Scope  NumInputPorts=3
  ksi_track_err_{1..5} (5 alike) : Scope  NumInputPorts=3
  leader control input : MATLAB Function  TreatAsAtomicUnit=on
  leader eta0 Integrator : Integrator  ExternalReset=rising  InitialConditionSource=external  InitialCondition=vel0
  leader ksi0 Integrator : Integrator  InitialCondition=pos0
  phi_{1..5} (5 alike) : Scope  NumInputPorts=3
  position observe Integrator {1..5} (5 alike) : Integrator  InitialCondition=zeros(3,1)
  process velocity : MATLAB Function  TreatAsAtomicUnit=on
  set desire formation configuration : MATLAB Function  TreatAsAtomicUnit=on
  sigma_bar_v_hat Integrator {1..5} (5 alike) : Integrator  InitialCondition=zeros(3,1)
  sigma_bar_v_tilt_{1..5} (5 alike) : Scope  NumInputPorts=3
  sigma_v Integrator {1..5} (5 alike) : Integrator  InitialCondition=zeros(3,1)
  trans to column1 : MATLAB Function  TreatAsAtomicUnit=on
  trans to column10 : MATLAB Function  TreatAsAtomicUnit=on
  trans to column11 : MATLAB Function  TreatAsAtomicUnit=on
  trans to column12 : MATLAB Function  TreatAsAtomicUnit=on
  trans to column13 : MATLAB Function  TreatAsAtomicUnit=on
  trans to column14 : MATLAB Function  TreatAsAtomicUnit=on
  trans to column15 : MATLAB Function  TreatAsAtomicUnit=on
  trans to column16 : MATLAB Function  TreatAsAtomicUnit=on
  trans to column17 : MATLAB Function  TreatAsAtomicUnit=on
  trans to column18 : MATLAB Function  TreatAsAtomicUnit=on
  trans to column19 : MATLAB Function  TreatAsAtomicUnit=on
  trans to column2 : MATLAB Function  TreatAsAtomicUnit=on
  trans to column20 : MATLAB Function  TreatAsAtomicUnit=on
  trans to column21 : MATLAB Function  TreatAsAtomicUnit=on
  trans to column22 : MATLAB Function  TreatAsAtomicUnit=on
  trans to column23 : MATLAB Function  TreatAsAtomicUnit=on
  trans to column24 : MATLAB Function  TreatAsAtomicUnit=on
  trans to column25 : MATLAB Function  TreatAsAtomicUnit=on
  trans to column26 : MATLAB Function  TreatAsAtomicUnit=on
  trans to column27 : MATLAB Function  TreatAsAtomicUnit=on
  trans to column28 : MATLAB Function  TreatAsAtomicUnit=on
  trans to column29 : MATLAB Function  TreatAsAtomicUnit=on
  trans to column3 : MATLAB Function  TreatAsAtomicUnit=on
  trans to column30 : MATLAB Function  TreatAsAtomicUnit=on
  trans to column31 : MATLAB Function  TreatAsAtomicUnit=on
  trans to column32 : MATLAB Function  TreatAsAtomicUnit=on
  trans to column33 : MATLAB Function  TreatAsAtomicUnit=on
  trans to column34 : MATLAB Function  TreatAsAtomicUnit=on
  trans to column35 : MATLAB Function  TreatAsAtomicUnit=on
  trans to column36 : MATLAB Function  TreatAsAtomicUnit=on
  trans to column37 : MATLAB Function  TreatAsAtomicUnit=on
  trans to column38 : MATLAB Function  TreatAsAtomicUnit=on
  trans to column39 : MATLAB Function  TreatAsAtomicUnit=on
  trans to column4 : MATLAB Function  TreatAsAtomicUnit=on
  trans to column40 : MATLAB Function  TreatAsAtomicUnit=on
  trans to column41 : MATLAB Function  TreatAsAtomicUnit=on
  trans to column42 : MATLAB Function  TreatAsAtomicUnit=on
  trans to column43 : MATLAB Function  TreatAsAtomicUnit=on
  trans to column44 : MATLAB Function  TreatAsAtomicUnit=on
  trans to column45 : MATLAB Function  TreatAsAtomicUnit=on
  trans to column46 : MATLAB Function  TreatAsAtomicUnit=on
  trans to column47 : MATLAB Function  TreatAsAtomicUnit=on
  trans to column48 : MATLAB Function  TreatAsAtomicUnit=on
  trans to column49 : MATLAB Function  TreatAsAtomicUnit=on
  trans to column5 : MATLAB Function  TreatAsAtomicUnit=on
  trans to column50 : MATLAB Function  TreatAsAtomicUnit=on
  trans to column51 : MATLAB Function  TreatAsAtomicUnit=on
  trans to column52 : MATLAB Function  TreatAsAtomicUnit=on
  trans to column53 : MATLAB Function  TreatAsAtomicUnit=on
  trans to column54 : MATLAB Function  TreatAsAtomicUnit=on
  trans to column55 : MATLAB Function  TreatAsAtomicUnit=on
  trans to column56 : MATLAB Function  TreatAsAtomicUnit=on
  trans to column57 : MATLAB Function  TreatAsAtomicUnit=on
  trans to column58 : MATLAB Function  TreatAsAtomicUnit=on
  trans to column59 : MATLAB Function  TreatAsAtomicUnit=on
  trans to column6 : MATLAB Function  TreatAsAtomicUnit=on
  trans to column60 : MATLAB Function  TreatAsAtomicUnit=on
  trans to column7 : MATLAB Function  TreatAsAtomicUnit=on
  trans to column8 : MATLAB Function  TreatAsAtomicUnit=on
  trans to column9 : MATLAB Function  TreatAsAtomicUnit=on
  uav translational dynamics agent 1 : MATLAB Function  TreatAsAtomicUnit=on
  uav translational dynamics agent 2 : MATLAB Function  TreatAsAtomicUnit=on
  uav translational dynamics agent 3 : MATLAB Function  TreatAsAtomicUnit=on
  uav translational dynamics agent 4 : MATLAB Function  TreatAsAtomicUnit=on
  uav translational dynamics agent 5 : MATLAB Function  TreatAsAtomicUnit=on
  velocity observe Integrator {1..5} (5 alike) : Integrator  InitialCondition=zeros(3,1)
  virtual velocity tracking item agent 1 : MATLAB Function  TreatAsAtomicUnit=on
  virtual velocity tracking item agent 2 : MATLAB Function  TreatAsAtomicUnit=on
  virtual velocity tracking item agent 3 : MATLAB Function  TreatAsAtomicUnit=on
  virtual velocity tracking item agent 4 : MATLAB Function  TreatAsAtomicUnit=on
  virtual velocity tracking item agent 5 : MATLAB Function  TreatAsAtomicUnit=on
  wires:
  [u0] -> To Workspace3/1
  [eta0] -> To Workspace4/1
  [ksi0] -> To Workspace5/1
  follower etai Integrator agent 1/1 -> [eta_1], follower ksii Integrator agent 1/1
  follower etai Integrator agent 2/1 -> [eta_2], follower ksii Integrator agent 2/1
  follower etai Integrator agent 3/1 -> [eta_3], follower ksii Integrator agent 3/1
  follower etai Integrator agent 4/1 -> [eta_4], follower ksii Integrator agent 4/1
  follower etai Integrator agent 5/1 -> [eta_5], follower ksii Integrator agent 5/1
  follower ksii Integrator agent 1/1 -> [ksi_1]
  follower ksii Integrator agent 2/1 -> [ksi_2]
  follower ksii Integrator agent 3/1 -> [ksi_3]
  follower ksii Integrator agent 4/1 -> [ksi_4]
  follower ksii Integrator agent 5/1 -> [ksi_5]
  [eta_1] -> combine formation control input/1(eta_1)
  [eta_2] -> combine formation control input/2(eta_2)
  [eta_3] -> combine formation control input/3(eta_3)
  [eta_4] -> combine formation control input/4(eta_4)
  [eta_5] -> combine formation control input/5(eta_5)
  [ksi_1] -> combine formation control input/6(ksi_1)
  [ksi_2] -> combine formation control input/7(ksi_2)
  [ksi_3] -> combine formation control input/8(ksi_3)
  [ksi_4] -> combine formation control input/9(ksi_4)
  [ksi_5] -> combine formation control input/10(ksi_5)
  [ksi_i_vec] -> follower tracking error agent 1/3(ksi_i_vec)
  [eta_i_vec] -> follower tracking error agent 1/4(eta_i_vec)
  [ksi0] -> follower tracking error agent 1/5(ksi0)
  [eta0] -> follower tracking error agent 1/6(eta0)
  follower tracking error agent 1/2(eta_track_err_1) -> Display13/1, Demux24/1, [eta_track_err_1]
  follower tracking error agent 1/1(ksi_track_err_1) -> Display12/1, Demux23/1, [ksi_track_err_1]
  [eta0] -> follower tracking error agent 2/6(eta0)
  [ksi0] -> follower tracking error agent 2/5(ksi0)
  [eta_i_vec] -> follower tracking error agent 2/4(eta_i_vec)
  follower tracking error agent 2/2(eta_track_err_2) -> Display15/1, Demux26/1, [eta_track_err_2]
  [ksi_i_vec] -> follower tracking error agent 2/3(ksi_i_vec)
  follower tracking error agent 2/1(ksi_track_err_2) -> Display14/1, Demux25/1, [ksi_track_err_2]
  follower tracking error agent 3/2(eta_track_err_3) -> Display17/1, Demux28/1, [eta_track_err_3]
  follower tracking error agent 3/1(ksi_track_err_3) -> Display16/1, Demux27/1, [ksi_track_err_3]
  [eta0] -> follower tracking error agent 3/6(eta0)
  [eta_i_vec] -> follower tracking error agent 3/4(eta_i_vec)
  [ksi_i_vec] -> follower tracking error agent 3/3(ksi_i_vec)
  [ksi0] -> follower tracking error agent 3/5(ksi0)
  [ksi_i_vec] -> follower tracking error agent 4/3(ksi_i_vec)
  [ksi0] -> follower tracking error agent 4/5(ksi0)
  [eta_i_vec] -> follower tracking error agent 4/4(eta_i_vec)
  [eta0] -> follower tracking error agent 4/6(eta0)
  follower tracking error agent 4/2(eta_track_err_4) -> Display19/1, Demux30/1, [eta_track_err_4]
  follower tracking error agent 4/1(ksi_track_err_4) -> Display18/1, Demux29/1, [ksi_track_err_4]
  follower tracking error agent 5/1(ksi_track_err_5) -> Display20/1, Demux31/1, [ksi_track_err_5]
  [ksi_i_vec] -> follower tracking error agent 5/3(ksi_i_vec)
  [eta0] -> follower tracking error agent 5/6(eta0)
  [ksi0] -> follower tracking error agent 5/5(ksi0)
  [eta_i_vec] -> follower tracking error agent 5/4(eta_i_vec)
  follower tracking error agent 5/2(eta_track_err_5) -> Display21/1, Demux32/1, [eta_track_err_5]
  [ksi_track_err_1] -> combine follower eta ksi/1(ksi_track_err_1)
  [ksi_track_err_2] -> combine follower eta ksi/2(ksi_track_err_2)
  [ksi_track_err_3] -> combine follower eta ksi/3(ksi_track_err_3)
  [ksi_track_err_4] -> combine follower eta ksi/4(ksi_track_err_4)
  [ksi_track_err_5] -> combine follower eta ksi/5(ksi_track_err_5)
  [eta_track_err_1] -> combine follower eta ksi/6(eta_track_err_1)
  [eta_track_err_2] -> combine follower eta ksi/7(eta_track_err_2)
  [eta_track_err_3] -> combine follower eta ksi/8(eta_track_err_3)
  [eta_track_err_4] -> combine follower eta ksi/9(eta_track_err_4)
  [eta_track_err_5] -> combine follower eta ksi/10(eta_track_err_5)
  combine follower eta ksi/1(ksi_track_err_vec) -> [ksi_track_err_vec]
  combine follower eta ksi/2(eta_track_err_vec) -> [eta_track_err_vec]
  [eta_i_vec] -> To Workspace7/1
  [ksi_i_vec] -> To Workspace8/1
  [ksi_track_err_vec] -> To Workspace9/1
  [eta_track_err_vec] -> To Workspace10/1
  Demux23/2 -> ksi_track_err_1/2
  Demux23/1 -> ksi_track_err_1/1
  Demux23/3 -> ksi_track_err_1/3
  Demux24/2 -> eta_track_err_1/2
  Demux24/1 -> eta_track_err_1/1
  Demux24/3 -> eta_track_err_1/3
  Demux25/2 -> ksi_track_err_2/2
  Demux25/1 -> ksi_track_err_2/1
  Demux25/3 -> ksi_track_err_2/3
  Demux26/1 -> eta_track_err_2/1
  Demux26/3 -> eta_track_err_2/3
  Demux26/2 -> eta_track_err_2/2
  Demux27/1 -> ksi_track_err_3/1
  Demux27/3 -> ksi_track_err_3/3
  Demux27/2 -> ksi_track_err_3/2
  Demux28/3 -> eta_track_err_3/3
  Demux28/2 -> eta_track_err_3/2
  Demux28/1 -> eta_track_err_3/1
  Demux29/3 -> ksi_track_err_4/3
  Demux29/2 -> ksi_track_err_4/2
  Demux29/1 -> ksi_track_err_4/1
  Demux30/3 -> eta_track_err_4/3
  Demux30/2 -> eta_track_err_4/2
  Demux30/1 -> eta_track_err_4/1
  Demux31/3 -> ksi_track_err_5/3
  Demux31/2 -> ksi_track_err_5/2
  Demux31/1 -> ksi_track_err_5/1
  Demux32/3 -> eta_track_err_5/3
  Demux32/2 -> eta_track_err_5/2
  Demux32/1 -> eta_track_err_5/1
  combine formation control input/1(eta_i_vec) -> Memory1/1
  Memory1/1 -> [eta_i_vec]
  combine formation control input/2(ksi_i_vec) -> Memory2/1
  Memory2/1 -> [ksi_i_vec]
  [ui_vec] -> To Workspace14/1
  [ui] -> uav translational dynamics agent 1/2(ui)
  [Ri] -> uav translational dynamics agent 1/1(Ri)
  uav translational dynamics agent 1/1(dvi) -> follower etai Integrator agent 1/1
  uav translational dynamics agent 2/1(dvi) -> follower etai Integrator agent 2/1
  [ui] -> uav translational dynamics agent 2/2(ui)
  [Ri] -> uav translational dynamics agent 2/1(Ri)
  [ui] -> uav translational dynamics agent 3/2(ui)
  [Ri] -> uav translational dynamics agent 3/1(Ri)
  uav translational dynamics agent 3/1(dvi) -> follower etai Integrator agent 3/1
  [ui] -> uav translational dynamics agent 4/2(ui)
  [Ri] -> uav translational dynamics agent 4/1(Ri)
  uav translational dynamics agent 4/1(dvi) -> follower etai Integrator agent 4/1
  [ui] -> uav translational dynamics agent 5/2(ui)
  [Ri] -> uav translational dynamics agent 5/1(Ri)
  uav translational dynamics agent 5/1(dvi) -> follower etai Integrator agent 5/1
  [ui] -> cal Rci from ui/2(ui)
  Constant191/1 -> cal Rci from ui/1(mi)
  cal Rei/1(Rei) -> depart Re5/1(x), depart Re4/1(x), depart Re3/1(x), depart Re2/1(x), depart Re1/1(x), [Rei]
  depart Re2/1(y) -> Display65/1
  depart Re3/1(y) -> Display66/1
  depart Re1/1(y) -> Display64/1
  depart Re4/1(y) -> Display67/1
  Constant51/1 -> cal Rei/1(Qei)
  depart Re5/1(y) -> Display68/1
  [Rei] -> cal Ri/1(Rei)
  [Rci] -> cal Ri/2(Rci)
  cal Ri/1(Ri) -> [Ri]
  depart Rc5/1(y) -> Display25/1
  depart Rc2/1(y) -> Display22/1
  depart Rc3/1(y) -> Display23/1
  depart Rc4/1(y) -> Display24/1
  depart Rc1/1(y) -> Display6/1
  cal Rci from ui/1(Rci) -> [Rci], depart Rc5/1(x), depart Rc4/1(x), depart Rc3/1(x), depart Rc2/1(x), depart Rc1/1(x)
  [tsim] -> generate translational disturbance agent 1/4(t)
  generate translational disturbance agent 1/1(dp_1) -> [dp_1]
  [dp_1] -> combine translational disturbance/1(dp_1)
  [dp_2] -> combine translational disturbance/2(dp_2)
  [dp_3] -> combine translational disturbance/3(dp_3)
  [dp_4] -> combine translational disturbance/4(dp_4)
  [dp_5] -> combine translational disturbance/5(dp_5)
  combine translational disturbance/1(dp_vec) -> [dp_vec]
  [dp_vec] -> uav translational dynamics agent 1/3(dp)
  [dp_vec] -> uav translational dynamics agent 2/3(dp)
  [dp_vec] -> uav translational dynamics agent 3/3(dp)
  [dp_vec] -> uav translational dynamics agent 4/3(dp)
  [dp_vec] -> uav translational dynamics agent 5/3(dp)
  Interpreted MATLAB Function1/1 -> trans to column1/1(x)
  Constant2/1 -> Mux30/2
  cal theta_err_ksi agent 1/1(theta_err_ksi_1_1) -> [theta_err_ksi_1_1]
  cal abs 2/1(y) -> Mux30/1
  choose ksi_est_err 1/1(y) -> cal abs 1/1(x)
  Constant3/1 -> Mux30/3
  [err_ksi_vec] -> choose ksi_est_err 2/1(x)
  [err_ksi_vec] -> choose ksi_est_err 1/1(x)
  cal abs 1/1(y) -> Mux36/1
  Interpreted MATLAB Function35/1 -> trans to column35/1(x)
  Constant1/1 -> Mux36/3
  Constant63/1 -> Mux36/2
  Mux36/1 -> Interpreted MATLAB Function35/1
  trans to column35/1(y) -> [err_ksi_squ_1_node_1], Display74/1
  cal theta_err_ksi agent 1/2(theta_err_ksi_2_1) -> [theta_err_ksi_2_1]
  trans to column1/1(y) -> [err_ksi_squ_2_node_1], Display1/1
  Mux30/1 -> Interpreted MATLAB Function1/1
  Constant16/1 -> cal theta_err_ksi agent 1/1(alfa_theta)
  [err_ksi_squ_2_node_1] -> cal theta_err_ksi agent 1/3(err_ksi_squ_2_node_1)
  choose ksi_est_err 2/1(y) -> cal abs 2/1(x)
  [err_ksi_squ_1_node_1] -> cal theta_err_ksi agent 1/2(err_ksi_squ_1_node_1)
  [err_ksi_vec] -> cal theta_err_ksi agent 1/4(err_ksi_vec)
  [err_ksi_vec] -> cal theta_err_ksi agent 2/4(err_ksi_vec)
  trans to column3/1(y) -> [err_ksi_squ_1_node_2], Display3/1
  Constant8/1 -> Mux2/2
  Constant4/1 -> Mux2/3
  Interpreted MATLAB Function3/1 -> trans to column3/1(x)
  [err_ksi_vec] -> choose ksi_est_err 3/1(x)
  [err_ksi_vec] -> choose ksi_est_err 4/1(x)
  choose ksi_est_err 3/1(y) -> cal abs 3/1(x)
  cal theta_err_ksi agent 2/1(theta_err_ksi_1_2) -> [theta_err_ksi_1_2]
  cal abs 4/1(y) -> Mux1/1
  Constant6/1 -> Mux1/2
  Interpreted MATLAB Function2/1 -> trans to column2/1(x)
  cal abs 3/1(y) -> Mux2/1
  choose ksi_est_err 4/1(y) -> cal abs 4/1(x)
  [err_ksi_squ_1_node_2] -> cal theta_err_ksi agent 2/2(err_ksi_squ_1_node_2)
  cal theta_err_ksi agent 2/2(theta_err_ksi_2_2) -> [theta_err_ksi_2_2]
  Mux1/1 -> Interpreted MATLAB Function2/1
  Constant5/1 -> cal theta_err_ksi agent 2/1(alfa_theta)
  trans to column2/1(y) -> [err_ksi_squ_2_node_2], Display2/1
  [err_ksi_squ_2_node_2] -> cal theta_err_ksi agent 2/3(err_ksi_squ_2_node_2)
  Constant7/1 -> Mux1/3
  Mux2/1 -> Interpreted MATLAB Function3/1
  [err_ksi_vec] -> choose ksi_est_err 6/1(x)
  Constant9/1 -> Mux4/3
  Constant13/1 -> Mux4/2
  trans to column5/1(y) -> [err_ksi_squ_1_node_3], Display5/1
  [err_ksi_vec] -> choose ksi_est_err 5/1(x)
  [err_ksi_vec] -> cal theta_err_ksi agent 3/4(err_ksi_vec)
  choose ksi_est_err 5/1(y) -> cal abs 5/1(x)
  [err_ksi_squ_2_node_3] -> cal theta_err_ksi agent 3/3(err_ksi_squ_2_node_3)
  trans to column4/1(y) -> [err_ksi_squ_2_node_3], Display4/1
  Mux4/1 -> Interpreted MATLAB Function5/1
  Constant10/1 -> cal theta_err_ksi agent 3/1(alfa_theta)
  Constant12/1 -> Mux3/3
  choose ksi_est_err 6/1(y) -> cal abs 6/1(x)
  Interpreted MATLAB Function5/1 -> trans to column5/1(x)
  [err_ksi_squ_1_node_3] -> cal theta_err_ksi agent 3/2(err_ksi_squ_1_node_3)
  cal theta_err_ksi agent 3/1(theta_err_ksi_1_3) -> [theta_err_ksi_1_3]
  cal abs 5/1(y) -> Mux4/1
  cal abs 6/1(y) -> Mux3/1
  Constant11/1 -> Mux3/2
  Interpreted MATLAB Function4/1 -> trans to column4/1(x)
  cal theta_err_ksi agent 3/2(theta_err_ksi_2_3) -> [theta_err_ksi_2_3]
  Mux3/1 -> Interpreted MATLAB Function4/1
  cal theta_err_ksi agent 4/2(theta_err_ksi_2_4) -> [theta_err_ksi_2_4]
  Constant15/1 -> Mux5/2
  Constant17/1 -> Mux5/3
  choose ksi_est_err 8/1(y) -> cal abs 8/1(x)
  cal abs 8/1(y) -> Mux5/1
  Constant14/1 -> cal theta_err_ksi agent 4/1(alfa_theta)
  cal theta_err_ksi agent 4/1(theta_err_ksi_1_4) -> [theta_err_ksi_1_4]
  [err_ksi_squ_1_node_4] -> cal theta_err_ksi agent 4/2(err_ksi_squ_1_node_4)
  cal abs 7/1(y) -> Mux6/1
  Interpreted MATLAB Function6/1 -> trans to column6/1(x)
  choose ksi_est_err 7/1(y) -> cal abs 7/1(x)
  [err_ksi_vec] -> cal theta_err_ksi agent 4/4(err_ksi_vec)
  trans to column6/1(y) -> [err_ksi_squ_2_node_4], Display7/1
  [err_ksi_squ_2_node_4] -> cal theta_err_ksi agent 4/3(err_ksi_squ_2_node_4)
  [err_ksi_vec] -> choose ksi_est_err 8/1(x)
  Mux5/1 -> Interpreted MATLAB Function6/1
  Constant18/1 -> Mux6/2
  trans to column7/1(y) -> [err_ksi_squ_1_node_4], Display8/1
  Interpreted MATLAB Function7/1 -> trans to column7/1(x)
  Mux6/1 -> Interpreted MATLAB Function7/1
  Constant19/1 -> Mux6/3
  [err_ksi_vec] -> choose ksi_est_err 7/1(x)
  Mux8/1 -> Interpreted MATLAB Function9/1
  Interpreted MATLAB Function9/1 -> trans to column9/1(x)
  [err_ksi_vec] -> choose ksi_est_err 9/1(x)
  Constant24/1 -> Mux8/3
  trans to column8/1(y) -> [err_ksi_squ_2_node_5], Display9/1
  Constant23/1 -> Mux8/2
  [err_ksi_squ_2_node_5] -> cal theta_err_ksi agent 5/3(err_ksi_squ_2_node_5)
  Mux7/1 -> Interpreted MATLAB Function8/1
  trans to column9/1(y) -> [err_ksi_squ_1_node_5], Display10/1
  choose ksi_est_err 9/1(y) -> cal abs 9/1(x)
  Interpreted MATLAB Function8/1 -> trans to column8/1(x)
  [err_ksi_vec] -> cal theta_err_ksi agent 5/4(err_ksi_vec)
  choose ksi_est_err 10/1(y) -> cal abs 10/1(x)
  [err_ksi_vec] -> choose ksi_est_err 10/1(x)
  [err_ksi_squ_1_node_5] -> cal theta_err_ksi agent 5/2(err_ksi_squ_1_node_5)
  cal abs 10/1(y) -> Mux7/1
  cal theta_err_ksi agent 5/1(theta_err_ksi_1_5) -> [theta_err_ksi_1_5]
  Constant22/1 -> Mux7/3
  Constant20/1 -> cal theta_err_ksi agent 5/1(alfa_theta)
  cal theta_err_ksi agent 5/2(theta_err_ksi_2_5) -> [theta_err_ksi_2_5]
  Constant21/1 -> Mux7/2
  cal abs 9/1(y) -> Mux8/1
  [theta_err_ksi_2_3] -> combine theta_err_ksi/8(theta_err_ksi_2_3)
  [theta_err_ksi_2_5] -> combine theta_err_ksi/10(theta_err_ksi_2_5)
  combine theta_err_ksi/2(theta_err_ksi_2_vec) -> [theta_err_ksi_2_vec]
  [theta_err_ksi_1_2] -> combine theta_err_ksi/2(theta_err_ksi_1_2)
  [theta_err_ksi_1_3] -> combine theta_err_ksi/3(theta_err_ksi_1_3)
  [theta_err_ksi_1_1] -> combine theta_err_ksi/1(theta_err_ksi_1_1)
  combine theta_err_ksi/1(theta_err_ksi_1_vec) -> [theta_err_ksi_1_vec]
  [theta_err_ksi_1_5] -> combine theta_err_ksi/5(theta_err_ksi_1_5)
  [theta_err_ksi_2_2] -> combine theta_err_ksi/7(theta_err_ksi_2_2)
  [theta_err_ksi_1_4] -> combine theta_err_ksi/4(theta_err_ksi_1_4)
  [theta_err_ksi_2_1] -> combine theta_err_ksi/6(theta_err_ksi_2_1)
  [theta_err_ksi_2_4] -> combine theta_err_ksi/9(theta_err_ksi_2_4)
  Constant26/1 -> virtual velocity tracking item agent 1/1(kai_chi_1)
  [theta_err_ksi_1_vec] -> virtual velocity tracking item agent 1/3(theta_err_ksi_1_vec)
  [theta_err_ksi_2_vec] -> virtual velocity tracking item agent 1/4(theta_err_ksi_2_vec)
  Constant25/1 -> virtual velocity tracking item agent 1/2(kai_chi_2)
  virtual velocity tracking item agent 1/1(chi_1) -> [chi_1]
  [theta_err_ksi_2_vec] -> virtual velocity tracking item agent 2/4(theta_err_ksi_2_vec)
  Constant28/1 -> virtual velocity tracking item agent 2/1(kai_chi_1)
  virtual velocity tracking item agent 2/1(chi_2) -> [chi_2]
  [theta_err_ksi_1_vec] -> virtual velocity tracking item agent 2/3(theta_err_ksi_1_vec)
  Constant27/1 -> virtual velocity tracking item agent 2/2(kai_chi_2)
  virtual velocity tracking item agent 3/1(chi_3) -> [chi_3]
  [theta_err_ksi_1_vec] -> virtual velocity tracking item agent 3/3(theta_err_ksi_1_vec)
  [theta_err_ksi_2_vec] -> virtual velocity tracking item agent 3/4(theta_err_ksi_2_vec)
  Constant29/1 -> virtual velocity tracking item agent 3/2(kai_chi_2)
  Constant30/1 -> virtual velocity tracking item agent 3/1(kai_chi_1)
  Constant32/1 -> virtual velocity tracking item agent 4/1(kai_chi_1)
  Constant31/1 -> virtual velocity tracking item agent 4/2(kai_chi_2)
  virtual velocity tracking item agent 4/1(chi_4) -> [chi_4]
  [theta_err_ksi_2_vec] -> virtual velocity tracking item agent 4/4(theta_err_ksi_2_vec)
  [theta_err_ksi_1_vec] -> virtual velocity tracking item agent 4/3(theta_err_ksi_1_vec)
  [theta_err_ksi_1_vec] -> virtual velocity tracking item agent 5/3(theta_err_ksi_1_vec)
  [theta_err_ksi_2_vec] -> virtual velocity tracking item agent 5/4(theta_err_ksi_2_vec)
  Constant34/1 -> virtual velocity tracking item agent 5/1(kai_chi_1)
  Constant33/1 -> virtual velocity tracking item agent 5/2(kai_chi_2)
  virtual velocity tracking item agent 5/1(chi_5) -> [chi_5]
  [chi_1] -> combine chi/1(chi_1)
  [chi_2] -> combine chi/2(chi_2)
  [chi_3] -> combine chi/3(chi_3)
  [chi_4] -> combine chi/4(chi_4)
  [chi_5] -> combine chi/5(chi_5)
  combine chi/1(chi_vec) -> [chi_vec]
  [err_eta_vec] -> cal virtual velocity control error phi/1(err_eta_vec)
  [chi_vec] -> cal virtual velocity control error phi/2(chi_vec)
  cal virtual velocity control error phi/1(phi_vec) -> [phi_vec]
  trans to column11/1(y) -> [d_err_ksi_squ_1_node_1], Display26/1
  Constant38/1 -> Mux10/2
  Constant35/1 -> Mux10/3
  Interpreted MATLAB Function11/1 -> trans to column11/1(x)
  [err_ksi_vec] -> choose ksi_est_err 11/1(x)
  [err_ksi_vec] -> choose ksi_est_err 12/1(x)
  choose ksi_est_err 11/1(y) -> cal abs 11/1(x)
  Constant36/1 -> Mux9/2
  cal abs 12/1(y) -> Mux9/1
  choose ksi_est_err 12/1(y) -> cal abs 12/1(x)
  Interpreted MATLAB Function10/1 -> trans to column10/1(x)
  cal abs 11/1(y) -> Mux10/1
  Mux9/1 -> Interpreted MATLAB Function10/1
  trans to column10/1(y) -> [d_err_ksi_squ_2_node_1], Display11/1
  Constant37/1 -> Mux9/3
  Mux10/1 -> Interpreted MATLAB Function11/1
  cal d_theta_err_ksi agent 1/1(d_theta_err_ksi_1_1) -> [d_theta_err_ksi_1_1]
  cal d_theta_err_ksi agent 1/2(d_theta_err_ksi_2_1) -> [d_theta_err_ksi_2_1]
  [err_ksi_vec] -> cal d_theta_err_ksi agent 1/8(err_ksi_vec)
  Constant39/1 -> cal d_theta_err_ksi agent 1/1(alfa_theta)
  [err_eta_vec] -> cal d_theta_err_ksi agent 1/9(err_eta_vec)
  [d_err_ksi_squ_2_node_1] -> cal d_theta_err_ksi agent 1/5(d_err_ksi_squ_2_node_1)
  [d_err_ksi_squ_1_node_1] -> cal d_theta_err_ksi agent 1/4(d_err_ksi_squ_1_node_1)
  Constant40/1 -> cal d_theta_err_ksi agent 1/2(beta1)
  Constant41/1 -> cal d_theta_err_ksi agent 1/3(beta2)
  [err_ksi_squ_2_node_1] -> cal d_theta_err_ksi agent 1/7(err_ksi_squ_2_node_1)
  [err_ksi_squ_1_node_1] -> cal d_theta_err_ksi agent 1/6(err_ksi_squ_1_node_1)
  [err_ksi_squ_1_node_2] -> cal d_theta_err_ksi agent 2/6(err_ksi_squ_1_node_2)
  Constant48/1 -> cal d_theta_err_ksi agent 2/3(beta2)
  [err_eta_vec] -> cal d_theta_err_ksi agent 2/9(err_eta_vec)
  Mux11/1 -> Interpreted MATLAB Function13/1
  [d_err_ksi_squ_1_node_2] -> cal d_theta_err_ksi agent 2/4(d_err_ksi_squ_1_node_2)
  Mux12/1 -> Interpreted MATLAB Function12/1
  Constant47/1 -> cal d_theta_err_ksi agent 2/2(beta1)
  Constant43/1 -> Mux12/2
  [err_ksi_vec] -> choose ksi_est_err 14/1(x)
  Interpreted MATLAB Function12/1 -> trans to column12/1(x)
  choose ksi_est_err 13/1(y) -> cal abs 13/1(x)
  cal abs 13/1(y) -> Mux11/1
  Constant44/1 -> Mux12/3
  choose ksi_est_err 14/1(y) -> cal abs 14/1(x)
  [d_err_ksi_squ_2_node_2] -> cal d_theta_err_ksi agent 2/5(d_err_ksi_squ_2_node_2)
  Constant45/1 -> Mux11/2
  Constant42/1 -> Mux11/3
  [err_ksi_vec] -> choose ksi_est_err 13/1(x)
  trans to column12/1(y) -> [d_err_ksi_squ_2_node_2], Display27/1
  Interpreted MATLAB Function13/1 -> trans to column13/1(x)
  cal abs 14/1(y) -> Mux12/1
  Constant46/1 -> cal d_theta_err_ksi agent 2/1(alfa_theta)
  cal d_theta_err_ksi agent 2/2(d_theta_err_ksi_2_2) -> [d_theta_err_ksi_2_2]
  cal d_theta_err_ksi agent 2/1(d_theta_err_ksi_1_2) -> [d_theta_err_ksi_1_2]
  [err_ksi_squ_2_node_2] -> cal d_theta_err_ksi agent 2/7(err_ksi_squ_2_node_2)
  [err_ksi_vec] -> cal d_theta_err_ksi agent 2/8(err_ksi_vec)
  trans to column13/1(y) -> [d_err_ksi_squ_1_node_2], Display28/1
  [err_ksi_squ_2_node_3] -> cal d_theta_err_ksi agent 3/7(err_ksi_squ_2_node_3)
  [err_ksi_vec] -> cal d_theta_err_ksi agent 3/8(err_ksi_vec)
  trans to column15/1(y) -> [d_err_ksi_squ_1_node_3], Display30/1
  cal abs 16/1(y) -> Mux14/1
  Constant54/1 -> cal d_theta_err_ksi agent 3/1(alfa_theta)
  cal d_theta_err_ksi agent 3/2(d_theta_err_ksi_2_3) -> [d_theta_err_ksi_2_3]
  Interpreted MATLAB Function15/1 -> trans to column15/1(x)
  cal d_theta_err_ksi agent 3/1(d_theta_err_ksi_1_3) -> [d_theta_err_ksi_1_3]
  Constant49/1 -> Mux13/3
  trans to column14/1(y) -> [d_err_ksi_squ_2_node_3], Display29/1
  [err_ksi_vec] -> choose ksi_est_err 15/1(x)
  Constant53/1 -> Mux13/2
  choose ksi_est_err 16/1(y) -> cal abs 16/1(x)
  choose ksi_est_err 15/1(y) -> cal abs 15/1(x)
  Constant52/1 -> Mux14/3
  cal abs 15/1(y) -> Mux13/1
  Interpreted MATLAB Function14/1 -> trans to column14/1(x)
  Constant55/1 -> cal d_theta_err_ksi agent 3/2(beta1)
  [d_err_ksi_squ_1_node_3] -> cal d_theta_err_ksi agent 3/4(d_err_ksi_squ_1_node_3)
  Constant56/1 -> cal d_theta_err_ksi agent 3/3(beta2)
  Mux13/1 -> Interpreted MATLAB Function15/1
  [d_err_ksi_squ_2_node_3] -> cal d_theta_err_ksi agent 3/5(d_err_ksi_squ_2_node_3)
  Constant50/1 -> Mux14/2
  [err_eta_vec] -> cal d_theta_err_ksi agent 3/9(err_eta_vec)
  Mux14/1 -> Interpreted MATLAB Function14/1
  [err_ksi_vec] -> choose ksi_est_err 16/1(x)
  [err_ksi_squ_1_node_3] -> cal d_theta_err_ksi agent 3/6(err_ksi_squ_1_node_3)
  [err_ksi_vec] -> choose ksi_est_err 18/1(x)
  Mux15/1 -> Interpreted MATLAB Function17/1
  Interpreted MATLAB Function16/1 -> trans to column16/1(x)
  [err_eta_vec] -> cal d_theta_err_ksi agent 4/9(err_eta_vec)
  Mux16/1 -> Interpreted MATLAB Function16/1
  Constant58/1 -> Mux16/2
  Constant62/1 -> cal d_theta_err_ksi agent 4/2(beta1)
  [d_err_ksi_squ_1_node_4] -> cal d_theta_err_ksi agent 4/4(d_err_ksi_squ_1_node_4)
  [d_err_ksi_squ_2_node_4] -> cal d_theta_err_ksi agent 4/5(d_err_ksi_squ_2_node_4)
  cal abs 17/1(y) -> Mux15/1
  [err_ksi_squ_1_node_4] -> cal d_theta_err_ksi agent 4/6(err_ksi_squ_1_node_4)
  trans to column16/1(y) -> [d_err_ksi_squ_2_node_4], Display31/1
  Constant59/1 -> Mux16/3
  Constant74/1 -> cal d_theta_err_ksi agent 4/3(beta2)
  choose ksi_est_err 17/1(y) -> cal abs 17/1(x)
  choose ksi_est_err 18/1(y) -> cal abs 18/1(x)
  Constant60/1 -> Mux15/2
  [err_ksi_vec] -> choose ksi_est_err 17/1(x)
  cal abs 18/1(y) -> Mux16/1
  Interpreted MATLAB Function17/1 -> trans to column17/1(x)
  Constant57/1 -> Mux15/3
  trans to column17/1(y) -> [d_err_ksi_squ_1_node_4], Display32/1
  cal d_theta_err_ksi agent 4/1(d_theta_err_ksi_1_4) -> [d_theta_err_ksi_1_4]
  [err_ksi_vec] -> cal d_theta_err_ksi agent 4/8(err_ksi_vec)
  Constant61/1 -> cal d_theta_err_ksi agent 4/1(alfa_theta)
  [err_ksi_squ_2_node_4] -> cal d_theta_err_ksi agent 4/7(err_ksi_squ_2_node_4)
  cal d_theta_err_ksi agent 4/2(d_theta_err_ksi_2_4) -> [d_theta_err_ksi_2_4]
  [d_err_ksi_squ_2_node_5] -> cal d_theta_err_ksi agent 5/5(d_err_ksi_squ_2_node_5)
  Constant80/1 -> cal d_theta_err_ksi agent 5/2(beta1)
  Constant76/1 -> Mux18/2
  [d_err_ksi_squ_1_node_5] -> cal d_theta_err_ksi agent 5/4(d_err_ksi_squ_1_node_5)
  Mux18/1 -> Interpreted MATLAB Function18/1
  Interpreted MATLAB Function18/1 -> trans to column18/1(x)
  [err_eta_vec] -> cal d_theta_err_ksi agent 5/9(err_eta_vec)
  cal d_theta_err_ksi agent 5/2(d_theta_err_ksi_2_5) -> [d_theta_err_ksi_2_5]
  [err_ksi_squ_2_node_5] -> cal d_theta_err_ksi agent 5/7(err_ksi_squ_2_node_5)
  [err_ksi_vec] -> choose ksi_est_err 20/1(x)
  [err_ksi_vec] -> cal d_theta_err_ksi agent 5/8(err_ksi_vec)
  trans to column19/1(y) -> [d_err_ksi_squ_1_node_5], Display34/1
  Constant79/1 -> cal d_theta_err_ksi agent 5/1(alfa_theta)
  Constant75/1 -> Mux17/3
  Interpreted MATLAB Function19/1 -> trans to column19/1(x)
  [err_ksi_vec] -> choose ksi_est_err 19/1(x)
  cal abs 20/1(y) -> Mux18/1
  Constant78/1 -> Mux17/2
  Constant77/1 -> Mux18/3
  choose ksi_est_err 20/1(y) -> cal abs 20/1(x)
  [err_ksi_squ_1_node_5] -> cal d_theta_err_ksi agent 5/6(err_ksi_squ_1_node_5)
  cal d_theta_err_ksi agent 5/1(d_theta_err_ksi_1_5) -> [d_theta_err_ksi_1_5]
  choose ksi_est_err 19/1(y) -> cal abs 19/1(x)
  Constant81/1 -> cal d_theta_err_ksi agent 5/3(beta2)
  Mux17/1 -> Interpreted MATLAB Function19/1
  trans to column18/1(y) -> [d_err_ksi_squ_2_node_5], Display33/1
  cal abs 19/1(y) -> Mux17/1
  [d_theta_err_ksi_2_vec] -> cal dchi agent 1/4(d_theta_err_ksi_2_vec)
  Constant83/1 -> cal dchi agent 1/1(kai_chi_1)
  cal dchi agent 1/1(d_chi_1) -> [d_chi_1]
  [d_theta_err_ksi_1_vec] -> cal dchi agent 1/3(d_theta_err_ksi_1_vec)
  Constant82/1 -> cal dchi agent 1/2(kai_chi_2)
  combine dtheta_err_ksi/1(d_theta_err_ksi_1_vec) -> [d_theta_err_ksi_1_vec]
  [d_theta_err_ksi_2_1] -> combine dtheta_err_ksi/6(d_theta_err_ksi_2_1)
  [d_theta_err_ksi_1_4] -> combine dtheta_err_ksi/4(d_theta_err_ksi_1_4)
  [d_theta_err_ksi_2_2] -> combine dtheta_err_ksi/7(d_theta_err_ksi_2_2)
  [d_theta_err_ksi_1_2] -> combine dtheta_err_ksi/2(d_theta_err_ksi_1_2)
  [d_theta_err_ksi_2_5] -> combine dtheta_err_ksi/10(d_theta_err_ksi_2_5)
  [d_theta_err_ksi_2_4] -> combine dtheta_err_ksi/9(d_theta_err_ksi_2_4)
  combine dtheta_err_ksi/2(d_theta_err_ksi_2_vec) -> [d_theta_err_ksi_2_vec]
  [d_theta_err_ksi_1_1] -> combine dtheta_err_ksi/1(d_theta_err_ksi_1_1)
  [d_theta_err_ksi_2_3] -> combine dtheta_err_ksi/8(d_theta_err_ksi_2_3)
  [d_theta_err_ksi_1_5] -> combine dtheta_err_ksi/5(d_theta_err_ksi_1_5)
  [d_theta_err_ksi_1_3] -> combine dtheta_err_ksi/3(d_theta_err_ksi_1_3)
  cal dchi agent 2/1(d_chi_2) -> [d_chi_2]
  [d_theta_err_ksi_1_vec] -> cal dchi agent 2/3(d_theta_err_ksi_1_vec)
  Constant85/1 -> cal dchi agent 2/1(kai_chi_1)
  Constant84/1 -> cal dchi agent 2/2(kai_chi_2)
  [d_theta_err_ksi_2_vec] -> cal dchi agent 2/4(d_theta_err_ksi_2_vec)
  [d_theta_err_ksi_2_vec] -> cal dchi agent 3/4(d_theta_err_ksi_2_vec)
  Constant87/1 -> cal dchi agent 3/1(kai_chi_1)
  [d_theta_err_ksi_1_vec] -> cal dchi agent 3/3(d_theta_err_ksi_1_vec)
  cal dchi agent 3/1(d_chi_3) -> [d_chi_3]
  Constant86/1 -> cal dchi agent 3/2(kai_chi_2)
  Constant88/1 -> cal dchi agent 4/2(kai_chi_2)
  Constant89/1 -> cal dchi agent 4/1(kai_chi_1)
  cal dchi agent 4/1(d_chi_4) -> [d_chi_4]
  [d_theta_err_ksi_1_vec] -> cal dchi agent 4/3(d_theta_err_ksi_1_vec)
  [d_theta_err_ksi_2_vec] -> cal dchi agent 4/4(d_theta_err_ksi_2_vec)
  Constant91/1 -> cal dchi agent 5/1(kai_chi_1)
  [d_theta_err_ksi_1_vec] -> cal dchi agent 5/3(d_theta_err_ksi_1_vec)
  cal dchi agent 5/1(d_chi_5) -> [d_chi_5]
  Constant90/1 -> cal dchi agent 5/2(kai_chi_2)
  [d_theta_err_ksi_2_vec] -> cal dchi agent 5/4(d_theta_err_ksi_2_vec)
  [d_chi_4] -> combine dchi/4(d_chi_4)
  combine dchi/1(d_chi_vec) -> [d_chi_vec]
  [d_chi_5] -> combine dchi/5(d_chi_5)
  [d_chi_2] -> combine dchi/2(d_chi_2)
  [d_chi_1] -> combine dchi/1(d_chi_1)
  [d_chi_3] -> combine dchi/3(d_chi_3)
  [Ri] -> cal virtual control sigma_v agent 1/2(Ri)
  [ui] -> cal virtual control sigma_v agent 1/3(ui_vec)
  Constant92/1 -> cal virtual control sigma_v agent 1/1(c3v)
  [sigma_bar_v_vec] -> cal virtual control sigma_v agent 1/4(sigma_bar_v_vec)
  cal virtual control sigma_v agent 1/1(d_sigma_v_1) -> sigma_v Integrator 1/1
  sigma_v Integrator 1/1 -> [sigma_v_1]
  [sigma_bar_v_vec] -> cal virtual control sigma_v agent 2/4(sigma_bar_v_vec)
  sigma_v Integrator 2/1 -> [sigma_v_2]
  Constant93/1 -> cal virtual control sigma_v agent 2/1(c3v)
  [Ri] -> cal virtual control sigma_v agent 2/2(Ri)
  cal virtual control sigma_v agent 2/1(d_sigma_v_2) -> sigma_v Integrator 2/1
  [ui] -> cal virtual control sigma_v agent 2/3(ui_vec)
  Constant94/1 -> cal virtual control sigma_v agent 3/1(c3v)
  cal virtual control sigma_v agent 3/1(d_sigma_v_3) -> sigma_v Integrator 3/1
  [ui] -> cal virtual control sigma_v agent 3/3(ui_vec)
  [Ri] -> cal virtual control sigma_v agent 3/2(Ri)
  [sigma_bar_v_vec] -> cal virtual control sigma_v agent 3/4(sigma_bar_v_vec)
  sigma_v Integrator 3/1 -> [sigma_v_3]
  sigma_v Integrator 4/1 -> [sigma_v_4]
  [Ri] -> cal virtual control sigma_v agent 4/2(Ri)
  [sigma_bar_v_vec] -> cal virtual control sigma_v agent 4/4(sigma_bar_v_vec)
  [ui] -> cal virtual control sigma_v agent 4/3(ui_vec)
  cal virtual control sigma_v agent 4/1(d_sigma_v_4) -> sigma_v Integrator 4/1
  Constant95/1 -> cal virtual control sigma_v agent 4/1(c3v)
  Constant96/1 -> cal virtual control sigma_v agent 5/1(c3v)
  [sigma_bar_v_vec] -> cal virtual control sigma_v agent 5/4(sigma_bar_v_vec)
  [Ri] -> cal virtual control sigma_v agent 5/2(Ri)
  [ui] -> cal virtual control sigma_v agent 5/3(ui_vec)
  sigma_v Integrator 5/1 -> [sigma_v_5]
  cal virtual control sigma_v agent 5/1(d_sigma_v_5) -> sigma_v Integrator 5/1
  combine sigma_v/1(sigma_v_vec) -> [sigma_v_vec]
  [sigma_v_4] -> combine sigma_v/4(sigma_v_4)
  [sigma_v_3] -> combine sigma_v/3(sigma_v_3)
  [sigma_v_1] -> combine sigma_v/1(sigma_v_1)
  [sigma_v_5] -> combine sigma_v/5(sigma_v_5)
  [sigma_v_2] -> combine sigma_v/2(sigma_v_2)
  [eta_i_vec] -> cal combine sigma_bar_v/1(eta_i_vec)
  [sigma_v_vec] -> cal combine sigma_bar_v/2(sigma_v_vec)
  cal combine sigma_bar_v/1(sigma_bar_v_vec) -> [sigma_bar_v_vec]
  Demux12/3 -> d2_sigma_bar_v_est_1/3
  Demux12/2 -> d2_sigma_bar_v_est_1/2
  Demux8/3 -> d_sigma_bar_v_est_1/3
  Demux12/1 -> d2_sigma_bar_v_est_1/1
  Demux8/1 -> d_sigma_bar_v_est_1/1
  Demux8/2 -> d_sigma_bar_v_est_1/2
  cal differentiator d_sigma_bar_v_hat agent 1/1(Out1) -> Display35/1, [sigma_bar_v_est_1]
  cal differentiator d_sigma_bar_v_hat agent 1/2(Out2) -> Demux8/1, [d_sigma_bar_v_est_1], Display36/1
  cal differentiator d_sigma_bar_v_hat agent 1/3(Out3) -> Demux12/1, [d2_sigma_bar_v_est_1], Display37/1
  [sigma_bar_v_vec] -> cal differentiator d_sigma_bar_v_hat agent 1/1(x)
  cal differentiator d_sigma_bar_v_hat agent 2/1(Out1) -> Display38/1, [sigma_bar_v_est_2]
  [sigma_bar_v_vec] -> cal differentiator d_sigma_bar_v_hat agent 2/1(x)
  cal differentiator d_sigma_bar_v_hat agent 2/2(Out2) -> Demux3/1, [d_sigma_bar_v_est_2], Display39/1
  cal differentiator d_sigma_bar_v_hat agent 2/3(Out3) -> Demux2/1, [d2_sigma_bar_v_est_2], Display40/1
  Demux2/2 -> d2_sigma_bar_v_est_2/2
  Demux2/3 -> d2_sigma_bar_v_est_2/3
  Demux3/2 -> d_sigma_bar_v_est_2/2
  Demux2/1 -> d2_sigma_bar_v_est_2/1
  Demux3/1 -> d_sigma_bar_v_est_2/1
  Demux3/3 -> d_sigma_bar_v_est_2/3
  Demux5/1 -> d_sigma_bar_v_est_3/1
  Demux5/3 -> d_sigma_bar_v_est_3/3
  Demux4/2 -> d2_sigma_bar_v_est_3/2
  Demux4/3 -> d2_sigma_bar_v_est_3/3
  Demux5/2 -> d_sigma_bar_v_est_3/2
  Demux4/1 -> d2_sigma_bar_v_est_3/1
  cal differentiator d_sigma_bar_v_hat agent 3/3(Out3) -> Demux4/1, [d2_sigma_bar_v_est_3], Display43/1
  cal differentiator d_sigma_bar_v_hat agent 3/2(Out2) -> Demux5/1, [d_sigma_bar_v_est_3], Display42/1
  cal differentiator d_sigma_bar_v_hat agent 3/1(Out1) -> Display41/1, [sigma_bar_v_est_3]
  [sigma_bar_v_vec] -> cal differentiator d_sigma_bar_v_hat agent 3/1(x)
  cal differentiator d_sigma_bar_v_hat agent 4/3(Out3) -> Demux6/1, [d2_sigma_bar_v_est_4], Display46/1
  Demux6/1 -> d2_sigma_bar_v_est_4/1
  Demux6/3 -> d2_sigma_bar_v_est_4/3
  Demux7/2 -> d_sigma_bar_v_est_4/2
  Demux6/2 -> d2_sigma_bar_v_est_4/2
  Demux7/3 -> d_sigma_bar_v_est_4/3
  Demux7/1 -> d_sigma_bar_v_est_4/1
  cal differentiator d_sigma_bar_v_hat agent 4/1(Out1) -> Display44/1, [sigma_bar_v_est_4]
  cal differentiator d_sigma_bar_v_hat agent 4/2(Out2) -> Demux7/1, [d_sigma_bar_v_est_4], Display45/1
  [sigma_bar_v_vec] -> cal differentiator d_sigma_bar_v_hat agent 4/1(x)
  cal differentiator d_sigma_bar_v_hat agent 5/1(Out1) -> Display47/1, [sigma_bar_v_est_5]
  cal differentiator d_sigma_bar_v_hat agent 5/2(Out2) -> Demux10/1, [d_sigma_bar_v_est_5], Display48/1
  [sigma_bar_v_vec] -> cal differentiator d_sigma_bar_v_hat agent 5/1(x)
  Demux10/3 -> d_sigma_bar_v_est_5/3
  Demux9/2 -> d2_sigma_bar_v_est_5/2
  Demux10/2 -> d_sigma_bar_v_est_5/2
  Demux9/1 -> d2_sigma_bar_v_est_5/1
  cal differentiator d_sigma_bar_v_hat agent 5/3(Out3) -> Demux9/1, [d2_sigma_bar_v_est_5], Display49/1
  Demux10/1 -> d_sigma_bar_v_est_5/1
  Demux9/3 -> d2_sigma_bar_v_est_5/3
  [d_sigma_bar_v_est_5] -> combine d_sigma_bar_v_est/5(d_sigma_bar_v_est_5)
  [d_sigma_bar_v_est_2] -> combine d_sigma_bar_v_est/2(d_sigma_bar_v_est_2)
  [d_sigma_bar_v_est_1] -> combine d_sigma_bar_v_est/1(d_sigma_bar_v_est_1)
  [d_sigma_bar_v_est_4] -> combine d_sigma_bar_v_est/4(d_sigma_bar_v_est_4)
  [d_sigma_bar_v_est_3] -> combine d_sigma_bar_v_est/3(d_sigma_bar_v_est_3)
  combine d_sigma_bar_v_est/1(d_sigma_bar_v_vec) -> [d_sigma_bar_v_vec]
  trans to column21/1(y) -> [sigma_bar_v_tilt_squ_1_1], Display51/1
  Constant100/1 -> Mux20/2
  Constant97/1 -> Mux20/3
  Interpreted MATLAB Function21/1 -> trans to column21/1(x)
  [sigma_bar_v_tilt_vec] -> choose ksi_est_err 21/1(x)
  choose ksi_est_err 21/1(y) -> cal abs 21/1(x)
  Constant98/1 -> Mux19/2
  cal abs 22/1(y) -> Mux19/1
  choose ksi_est_err 22/1(y) -> cal abs 22/1(x)
  Interpreted MATLAB Function20/1 -> trans to column20/1(x)
  cal abs 21/1(y) -> Mux20/1
  Mux19/1 -> Interpreted MATLAB Function20/1
  trans to column20/1(y) -> [sigma_bar_v_tilt_squ_2_1], Display50/1
  Constant99/1 -> Mux19/3
  Mux20/1 -> Interpreted MATLAB Function21/1
  [sigma_bar_v_tilt_vec] -> choose ksi_est_err 22/1(x)
  cal theta_sigma_bar_v_tilt agent 1/1(theta_sigma_bar_v_tilt_1_1) -> [theta_sigma_bar_v_tilt_1_1]
  [sigma_bar_v_tilt_squ_1_1] -> cal theta_sigma_bar_v_tilt agent 1/2(sigma_bar_v_tilt_squ_1_1)
  cal theta_sigma_bar_v_tilt agent 1/2(theta_sigma_bar_v_tilt_2_1) -> [theta_sigma_bar_v_tilt_2_1]
  [sigma_bar_v_tilt_vec] -> cal theta_sigma_bar_v_tilt agent 1/4(sigma_bar_v_tilt_vec)
  [sigma_bar_v_tilt_squ_2_1] -> cal theta_sigma_bar_v_tilt agent 1/3(sigma_bar_v_tilt_squ_2_1)
  Constant101/1 -> cal theta_sigma_bar_v_tilt agent 1/1(alfa_theta)
  Constant103/1 -> cal theta_sigma_bar_v_tilt agent 2/1(alfa_theta)
  [sigma_bar_v_tilt_vec] -> cal theta_sigma_bar_v_tilt agent 2/4(sigma_bar_v_tilt_vec)
  [sigma_bar_v_tilt_squ_1_2] -> cal theta_sigma_bar_v_tilt agent 2/2(sigma_bar_v_tilt_squ_1_2)
  trans to column23/1(y) -> [sigma_bar_v_tilt_squ_1_2], Display53/1
  Interpreted MATLAB Function23/1 -> trans to column23/1(x)
  Mux22/1 -> Interpreted MATLAB Function23/1
  Constant106/1 -> Mux21/3
  cal theta_sigma_bar_v_tilt agent 2/1(theta_sigma_bar_v_tilt_1_2) -> [theta_sigma_bar_v_tilt_1_2]
  Constant102/1 -> Mux22/2
  trans to column22/1(y) -> [sigma_bar_v_tilt_squ_2_2], Display52/1
  Interpreted MATLAB Function22/1 -> trans to column22/1(x)
  cal abs 23/1(y) -> Mux22/1
  Constant104/1 -> Mux22/3
  Mux21/1 -> Interpreted MATLAB Function22/1
  choose ksi_est_err 24/1(y) -> cal abs 24/1(x)
  cal abs 24/1(y) -> Mux21/1
  choose ksi_est_err 23/1(y) -> cal abs 23/1(x)
  [sigma_bar_v_tilt_vec] -> choose ksi_est_err 24/1(x)
  [sigma_bar_v_tilt_squ_2_2] -> cal theta_sigma_bar_v_tilt agent 2/3(sigma_bar_v_tilt_squ_2_2)
  Constant105/1 -> Mux21/2
  [sigma_bar_v_tilt_vec] -> choose ksi_est_err 23/1(x)
  cal theta_sigma_bar_v_tilt agent 2/2(theta_sigma_bar_v_tilt_2_2) -> [theta_sigma_bar_v_tilt_2_2]
  [sigma_bar_v_tilt_vec] -> choose ksi_est_err 25/1(x)
  cal theta_sigma_bar_v_tilt agent 3/2(theta_sigma_bar_v_tilt_2_3) -> [theta_sigma_bar_v_tilt_2_3]
  Constant110/1 -> Mux23/2
  [sigma_bar_v_tilt_squ_2_3] -> cal theta_sigma_bar_v_tilt agent 3/3(sigma_bar_v_tilt_squ_2_3)
  [sigma_bar_v_tilt_vec] -> choose ksi_est_err 26/1(x)
  choose ksi_est_err 25/1(y) -> cal abs 25/1(x)
  Mux23/1 -> Interpreted MATLAB Function24/1
  choose ksi_est_err 26/1(y) -> cal abs 26/1(x)
  Constant109/1 -> Mux24/3
  cal abs 25/1(y) -> Mux24/1
  Interpreted MATLAB Function24/1 -> trans to column24/1(x)
  Constant107/1 -> Mux24/2
  Mux24/1 -> Interpreted MATLAB Function25/1
  cal theta_sigma_bar_v_tilt agent 3/1(theta_sigma_bar_v_tilt_1_3) -> [theta_sigma_bar_v_tilt_1_3]
  Constant111/1 -> Mux23/3
  Constant108/1 -> cal theta_sigma_bar_v_tilt agent 3/1(alfa_theta)
  trans to column24/1(y) -> [sigma_bar_v_tilt_squ_2_3], Display54/1
  [sigma_bar_v_tilt_squ_1_3] -> cal theta_sigma_bar_v_tilt agent 3/2(sigma_bar_v_tilt_squ_1_3)
  trans to column25/1(y) -> [sigma_bar_v_tilt_squ_1_3], Display55/1
  Interpreted MATLAB Function25/1 -> trans to column25/1(x)
  [sigma_bar_v_tilt_vec] -> cal theta_sigma_bar_v_tilt agent 3/4(sigma_bar_v_tilt_vec)
  cal abs 26/1(y) -> Mux23/1
  cal abs 28/1(y) -> Mux25/1
  trans to column27/1(y) -> [sigma_bar_v_tilt_squ_1_4], Display57/1
  Interpreted MATLAB Function27/1 -> trans to column27/1(x)
  Constant113/1 -> cal theta_sigma_bar_v_tilt agent 4/1(alfa_theta)
  [sigma_bar_v_tilt_squ_1_4] -> cal theta_sigma_bar_v_tilt agent 4/2(sigma_bar_v_tilt_squ_1_4)
  Constant116/1 -> Mux25/3
  trans to column26/1(y) -> [sigma_bar_v_tilt_squ_2_4], Display56/1
  Constant112/1 -> Mux26/2
  Mux26/1 -> Interpreted MATLAB Function27/1
  [sigma_bar_v_tilt_vec] -> cal theta_sigma_bar_v_tilt agent 4/4(sigma_bar_v_tilt_vec)
  Constant114/1 -> Mux26/3
  cal abs 27/1(y) -> Mux26/1
  cal theta_sigma_bar_v_tilt agent 4/1(theta_sigma_bar_v_tilt_1_4) -> [theta_sigma_bar_v_tilt_1_4]
  Constant115/1 -> Mux25/2
  choose ksi_est_err 27/1(y) -> cal abs 27/1(x)
  choose ksi_est_err 28/1(y) -> cal abs 28/1(x)
  Interpreted MATLAB Function26/1 -> trans to column26/1(x)
  cal theta_sigma_bar_v_tilt agent 4/2(theta_sigma_bar_v_tilt_2_4) -> [theta_sigma_bar_v_tilt_2_4]
  [sigma_bar_v_tilt_vec] -> choose ksi_est_err 28/1(x)
  [sigma_bar_v_tilt_squ_2_4] -> cal theta_sigma_bar_v_tilt agent 4/3(sigma_bar_v_tilt_squ_2_4)
  [sigma_bar_v_tilt_vec] -> choose ksi_est_err 27/1(x)
  Mux25/1 -> Interpreted MATLAB Function26/1
  [sigma_bar_v_tilt_squ_2_5] -> cal theta_sigma_bar_v_tilt agent 5/3(sigma_bar_v_tilt_squ_2_5)
  choose ksi_est_err 29/1(y) -> cal abs 29/1(x)
  Interpreted MATLAB Function28/1 -> trans to column28/1(x)
  choose ksi_est_err 30/1(y) -> cal abs 30/1(x)
  Constant120/1 -> Mux27/2
  cal theta_sigma_bar_v_tilt agent 5/2(theta_sigma_bar_v_tilt_2_5) -> [theta_sigma_bar_v_tilt_2_5]
  [sigma_bar_v_tilt_vec] -> choose ksi_est_err 29/1(x)
  cal theta_sigma_bar_v_tilt agent 5/1(theta_sigma_bar_v_tilt_1_5) -> [theta_sigma_bar_v_tilt_1_5]
  [sigma_bar_v_tilt_vec] -> choose ksi_est_err 30/1(x)
  Constant119/1 -> Mux28/3
  trans to column28/1(y) -> [sigma_bar_v_tilt_squ_2_5], Display58/1
  Mux28/1 -> Interpreted MATLAB Function29/1
  Constant117/1 -> Mux28/2
  cal abs 29/1(y) -> Mux28/1
  [sigma_bar_v_tilt_squ_1_5] -> cal theta_sigma_bar_v_tilt agent 5/2(sigma_bar_v_tilt_squ_1_5)
  Mux27/1 -> Interpreted MATLAB Function28/1
  Constant121/1 -> Mux27/3
  Interpreted MATLAB Function29/1 -> trans to column29/1(x)
  [sigma_bar_v_tilt_vec] -> cal theta_sigma_bar_v_tilt agent 5/4(sigma_bar_v_tilt_vec)
  Constant118/1 -> cal theta_sigma_bar_v_tilt agent 5/1(alfa_theta)
  trans to column29/1(y) -> [sigma_bar_v_tilt_squ_1_5], Display59/1
  cal abs 30/1(y) -> Mux27/1
  combine theta_sigma_bar_v_tilt/1(theta_sigma_bar_v_tilt_1_vec) -> [theta_sigma_bar_v_tilt_1_vec]
  [theta_sigma_bar_v_tilt_2_1] -> combine theta_sigma_bar_v_tilt/6(theta_sigma_bar_v_tilt_2_1)
  [theta_sigma_bar_v_tilt_1_4] -> combine theta_sigma_bar_v_tilt/4(theta_sigma_bar_v_tilt_1_4)
  [theta_sigma_bar_v_tilt_2_2] -> combine theta_sigma_bar_v_tilt/7(theta_sigma_bar_v_tilt_2_2)
  [theta_sigma_bar_v_tilt_1_2] -> combine theta_sigma_bar_v_tilt/2(theta_sigma_bar_v_tilt_1_2)
  [theta_sigma_bar_v_tilt_2_5] -> combine theta_sigma_bar_v_tilt/10(theta_sigma_bar_v_tilt_2_5)
  [theta_sigma_bar_v_tilt_2_4] -> combine theta_sigma_bar_v_tilt/9(theta_sigma_bar_v_tilt_2_4)
  combine theta_sigma_bar_v_tilt/2(theta_sigma_bar_v_tilt_2_vec) -> [theta_sigma_bar_v_tilt_2_vec]
  [theta_sigma_bar_v_tilt_1_1] -> combine theta_sigma_bar_v_tilt/1(theta_sigma_bar_v_tilt_1_1)
  [theta_sigma_bar_v_tilt_2_3] -> combine theta_sigma_bar_v_tilt/8(theta_sigma_bar_v_tilt_2_3)
  [theta_sigma_bar_v_tilt_1_5] -> combine theta_sigma_bar_v_tilt/5(theta_sigma_bar_v_tilt_1_5)
  [theta_sigma_bar_v_tilt_1_3] -> combine theta_sigma_bar_v_tilt/3(theta_sigma_bar_v_tilt_1_3)
  Constant122/1 -> cal sigma_bar_v_hat agent 1/1(c1v)
  Constant123/1 -> cal sigma_bar_v_hat agent 1/2(c2v)
  [theta_sigma_bar_v_tilt_1_vec] -> cal sigma_bar_v_hat agent 1/3(theta_sigma_bar_v_tilt_1_vec)
  [theta_sigma_bar_v_tilt_2_vec] -> cal sigma_bar_v_hat agent 1/4(theta_sigma_bar_v_tilt_2_vec)
  [d_sigma_bar_v_vec] -> cal sigma_bar_v_hat agent 1/5(d_sigma_bar_v_vec)
  cal sigma_bar_v_hat agent 1/1(d_sigma_bar_v_hat_1) -> sigma_bar_v_hat Integrator 1/1
  [theta_sigma_bar_v_tilt_2_vec] -> cal sigma_bar_v_hat agent 2/4(theta_sigma_bar_v_tilt_2_vec)
  Constant125/1 -> cal sigma_bar_v_hat agent 2/2(c2v)
  cal sigma_bar_v_hat agent 2/1(d_sigma_bar_v_hat_2) -> sigma_bar_v_hat Integrator 2/1
  [d_sigma_bar_v_vec] -> cal sigma_bar_v_hat agent 2/5(d_sigma_bar_v_vec)
  [theta_sigma_bar_v_tilt_1_vec] -> cal sigma_bar_v_hat agent 2/3(theta_sigma_bar_v_tilt_1_vec)
  Constant124/1 -> cal sigma_bar_v_hat agent 2/1(c1v)
  Constant126/1 -> cal sigma_bar_v_hat agent 3/1(c1v)
  [theta_sigma_bar_v_tilt_2_vec] -> cal sigma_bar_v_hat agent 3/4(theta_sigma_bar_v_tilt_2_vec)
  cal sigma_bar_v_hat agent 3/1(d_sigma_bar_v_hat_3) -> sigma_bar_v_hat Integrator 3/1
  [d_sigma_bar_v_vec] -> cal sigma_bar_v_hat agent 3/5(d_sigma_bar_v_vec)
  Constant127/1 -> cal sigma_bar_v_hat agent 3/2(c2v)
  [theta_sigma_bar_v_tilt_1_vec] -> cal sigma_bar_v_hat agent 3/3(theta_sigma_bar_v_tilt_1_vec)
  [d_sigma_bar_v_vec] -> cal sigma_bar_v_hat agent 4/5(d_sigma_bar_v_vec)
  [theta_sigma_bar_v_tilt_1_vec] -> cal sigma_bar_v_hat agent 4/3(theta_sigma_bar_v_tilt_1_vec)
  Constant139/1 -> cal sigma_bar_v_hat agent 4/2(c2v)
  cal sigma_bar_v_hat agent 4/1(d_sigma_bar_v_hat_4) -> sigma_bar_v_hat Integrator 4/1
  [theta_sigma_bar_v_tilt_2_vec] -> cal sigma_bar_v_hat agent 4/4(theta_sigma_bar_v_tilt_2_vec)
  Constant128/1 -> cal sigma_bar_v_hat agent 4/1(c1v)
  [sigma_bar_v_hat_5] -> combine sigma_bar_v_hat/5(sigma_bar_v_hat_5)
  [sigma_bar_v_hat_4] -> combine sigma_bar_v_hat/4(sigma_bar_v_hat_4)
  [sigma_bar_v_hat_3] -> combine sigma_bar_v_hat/3(sigma_bar_v_hat_3)
  combine sigma_bar_v_hat/1(sigma_bar_v_hat_vec) -> [sigma_bar_v_hat_vec]
  cal combine sigma_bar_v_tilt/1(sigma_bar_v_tilt_vec) -> [sigma_bar_v_tilt_vec]
  [sigma_bar_v_vec] -> cal combine sigma_bar_v_tilt/1(sigma_bar_v_vec)
  [sigma_bar_v_hat_vec] -> cal combine sigma_bar_v_tilt/2(sigma_bar_v_hat_vec)
  [sigma_bar_v_hat_2] -> combine sigma_bar_v_hat/2(sigma_bar_v_hat_2)
  [sigma_bar_v_hat_1] -> combine sigma_bar_v_hat/1(sigma_bar_v_hat_1)
  sigma_bar_v_hat Integrator 1/1 -> [sigma_bar_v_hat_1]
  sigma_bar_v_hat Integrator 2/1 -> [sigma_bar_v_hat_2]
  sigma_bar_v_hat Integrator 3/1 -> [sigma_bar_v_hat_3]
  sigma_bar_v_hat Integrator 4/1 -> [sigma_bar_v_hat_4]
  sigma_bar_v_hat Integrator 5/1 -> [sigma_bar_v_hat_5]
  [d_sigma_bar_v_vec] -> cal sigma_bar_v_hat agent 5/5(d_sigma_bar_v_vec)
  [theta_sigma_bar_v_tilt_2_vec] -> cal sigma_bar_v_hat agent 5/4(theta_sigma_bar_v_tilt_2_vec)
  cal sigma_bar_v_hat agent 5/1(d_sigma_bar_v_hat_5) -> sigma_bar_v_hat Integrator 5/1
  [theta_sigma_bar_v_tilt_1_vec] -> cal sigma_bar_v_hat agent 5/3(theta_sigma_bar_v_tilt_1_vec)
  Constant141/1 -> cal sigma_bar_v_hat agent 5/2(c2v)
  Constant140/1 -> cal sigma_bar_v_hat agent 5/1(c1v)
  Constant142/1 -> cal dp_hat agent 1/1(c3v)
  [d_sigma_bar_v_vec] -> cal dp_hat agent 1/2(d_sigma_bar_v_vec)
  [sigma_bar_v_hat_vec] -> cal dp_hat agent 1/3(sigma_bar_v_hat_vec)
  cal dp_hat agent 1/1(dp_hat_1) -> [dp_hat_1]
  cal dp_hat agent 2/1(dp_hat_2) -> [dp_hat_2]
  [d_sigma_bar_v_vec] -> cal dp_hat agent 2/2(d_sigma_bar_v_vec)
  Constant143/1 -> cal dp_hat agent 2/1(c3v)
  [sigma_bar_v_hat_vec] -> cal dp_hat agent 2/3(sigma_bar_v_hat_vec)
  [sigma_bar_v_hat_vec] -> cal dp_hat agent 3/3(sigma_bar_v_hat_vec)
  Constant144/1 -> cal dp_hat agent 3/1(c3v)
  [d_sigma_bar_v_vec] -> cal dp_hat agent 3/2(d_sigma_bar_v_vec)
  cal dp_hat agent 3/1(dp_hat_3) -> [dp_hat_3]
  cal dp_hat agent 4/1(dp_hat_4) -> [dp_hat_4]
  [d_sigma_bar_v_vec] -> cal dp_hat agent 4/2(d_sigma_bar_v_vec)
  Constant145/1 -> cal dp_hat agent 4/1(c3v)
  [sigma_bar_v_hat_vec] -> cal dp_hat agent 4/3(sigma_bar_v_hat_vec)
  cal dp_hat agent 5/1(dp_hat_5) -> [dp_hat_5]
  [sigma_bar_v_hat_vec] -> cal dp_hat agent 5/3(sigma_bar_v_hat_vec)
  Constant146/1 -> cal dp_hat agent 5/1(c3v)
  [d_sigma_bar_v_vec] -> cal dp_hat agent 5/2(d_sigma_bar_v_vec)
  combine dp_hat/1(dp_hat_vec) -> [dp_hat_vec]
  [dp_hat_1] -> combine dp_hat/1(dp_hat_1)
  [dp_hat_4] -> combine dp_hat/4(dp_hat_4)
  [dp_hat_3] -> combine dp_hat/3(dp_hat_3)
  [dp_hat_5] -> combine dp_hat/5(dp_hat_5)
  [dp_hat_2] -> combine dp_hat/2(dp_hat_2)
  Constant148/1 -> cal theta_phi agent 1/1(alfa_theta)
  [phi_vec] -> cal theta_phi agent 1/4(phi_vec)
  [phi_squ_1_1] -> cal theta_phi agent 1/2(phi_squ_1_1)
  trans to column31/1(y) -> [phi_squ_1_1], Display61/1
  Interpreted MATLAB Function31/1 -> trans to column31/1(x)
  Mux31/1 -> Interpreted MATLAB Function31/1
  Constant151/1 -> Mux29/3
  cal theta_phi agent 1/1(theta_phi_1_1) -> [theta_phi_1_1]
  Constant147/1 -> Mux31/2
  trans to column30/1(y) -> [phi_squ_2_1], Display60/1
  Interpreted MATLAB Function30/1 -> trans to column30/1(x)
  cal abs 31/1(y) -> Mux31/1
  Constant149/1 -> Mux31/3
  Mux29/1 -> Interpreted MATLAB Function30/1
  choose ksi_est_err 32/1(y) -> cal abs 32/1(x)
  cal abs 32/1(y) -> Mux29/1
  choose ksi_est_err 31/1(y) -> cal abs 31/1(x)
  [phi_vec] -> choose ksi_est_err 32/1(x)
  [phi_squ_2_1] -> cal theta_phi agent 1/3(phi_squ_2_1)
  Constant150/1 -> Mux29/2
  [phi_vec] -> choose ksi_est_err 31/1(x)
  cal theta_phi agent 1/2(theta_phi_2_1) -> [theta_phi_2_1]
  cal theta_phi agent 2/2(theta_phi_2_2) -> [theta_phi_2_2]
  [phi_vec] -> choose ksi_est_err 33/1(x)
  [phi_squ_2_2] -> cal theta_phi agent 2/3(phi_squ_2_2)
  cal abs 34/1(y) -> Mux32/1
  choose ksi_est_err 34/1(y) -> cal abs 34/1(x)
  Constant154/1 -> Mux33/3
  Mux32/1 -> Interpreted MATLAB Function32/1
  Constant155/1 -> Mux32/2
  trans to column32/1(y) -> [phi_squ_2_2], Display62/1
  cal abs 33/1(y) -> Mux33/1
  [phi_vec] -> choose ksi_est_err 34/1(x)
  Interpreted MATLAB Function32/1 -> trans to column32/1(x)
  Constant152/1 -> Mux33/2
  cal theta_phi agent 2/1(theta_phi_1_2) -> [theta_phi_1_2]
  choose ksi_est_err 33/1(y) -> cal abs 33/1(x)
  [phi_squ_1_2] -> cal theta_phi agent 2/2(phi_squ_1_2)
  Interpreted MATLAB Function33/1 -> trans to column33/1(x)
  Constant156/1 -> Mux32/3
  [phi_vec] -> cal theta_phi agent 2/4(phi_vec)
  Mux33/1 -> Interpreted MATLAB Function33/1
  trans to column33/1(y) -> [phi_squ_1_2], Display63/1
  Constant153/1 -> cal theta_phi agent 2/1(alfa_theta)
  Constant158/1 -> cal theta_phi agent 3/1(alfa_theta)
  trans to column36/1(y) -> [phi_squ_1_3], Display70/1
  Interpreted MATLAB Function36/1 -> trans to column36/1(x)
  [phi_vec] -> cal theta_phi agent 3/4(phi_vec)
  [phi_squ_1_3] -> cal theta_phi agent 3/2(phi_squ_1_3)
  cal theta_phi agent 3/1(theta_phi_1_3) -> [theta_phi_1_3]
  choose ksi_est_err 35/1(y) -> cal abs 35/1(x)
  Mux35/1 -> Interpreted MATLAB Function36/1
  Constant161/1 -> Mux34/3
  [phi_vec] -> choose ksi_est_err 36/1(x)
  trans to column34/1(y) -> [phi_squ_2_3], Display69/1
  Interpreted MATLAB Function34/1 -> trans to column34/1(x)
  Constant157/1 -> Mux35/2
  cal abs 35/1(y) -> Mux35/1
  [phi_vec] -> choose ksi_est_err 35/1(x)
  choose ksi_est_err 36/1(y) -> cal abs 36/1(x)
  [phi_squ_2_3] -> cal theta_phi agent 3/3(phi_squ_2_3)
  Mux34/1 -> Interpreted MATLAB Function34/1
  Constant159/1 -> Mux35/3
  cal abs 36/1(y) -> Mux34/1
  cal theta_phi agent 3/2(theta_phi_2_3) -> [theta_phi_2_3]
  Constant160/1 -> Mux34/2
  choose ksi_est_err 38/1(y) -> cal abs 38/1(x)
  cal abs 37/1(y) -> Mux38/1
  [phi_vec] -> choose ksi_est_err 37/1(x)
  Mux37/1 -> Interpreted MATLAB Function37/1
  [phi_squ_2_4] -> cal theta_phi agent 4/3(phi_squ_2_4)
  Constant165/1 -> Mux37/2
  cal theta_phi agent 4/2(theta_phi_2_4) -> [theta_phi_2_4]
  cal abs 38/1(y) -> Mux37/1
  Interpreted MATLAB Function37/1 -> trans to column37/1(x)
  Constant164/1 -> Mux38/3
  [phi_vec] -> choose ksi_est_err 38/1(x)
  trans to column37/1(y) -> [phi_squ_2_4], Display71/1
  Constant162/1 -> Mux38/2
  [phi_vec] -> cal theta_phi agent 4/4(phi_vec)
  Mux38/1 -> Interpreted MATLAB Function38/1
  choose ksi_est_err 37/1(y) -> cal abs 37/1(x)
  Constant163/1 -> cal theta_phi agent 4/1(alfa_theta)
  Constant166/1 -> Mux37/3
  [phi_squ_1_4] -> cal theta_phi agent 4/2(phi_squ_1_4)
  cal theta_phi agent 4/1(theta_phi_1_4) -> [theta_phi_1_4]
  Interpreted MATLAB Function38/1 -> trans to column38/1(x)
  trans to column38/1(y) -> [phi_squ_1_4], Display72/1
  trans to column40/1(y) -> [phi_squ_1_5], Display75/1
  Interpreted MATLAB Function40/1 -> trans to column40/1(x)
  choose ksi_est_err 39/1(y) -> cal abs 39/1(x)
  Constant171/1 -> Mux39/3
  [phi_vec] -> cal theta_phi agent 5/4(phi_vec)
  [phi_squ_1_5] -> cal theta_phi agent 5/2(phi_squ_1_5)
  Constant168/1 -> cal theta_phi agent 5/1(alfa_theta)
  cal theta_phi agent 5/1(theta_phi_1_5) -> [theta_phi_1_5]
  Mux40/1 -> Interpreted MATLAB Function40/1
  Interpreted MATLAB Function39/1 -> trans to column39/1(x)
  Constant169/1 -> Mux40/3
  cal theta_phi agent 5/2(theta_phi_2_5) -> [theta_phi_2_5]
  Constant167/1 -> Mux40/2
  trans to column39/1(y) -> [phi_squ_2_5], Display73/1
  [phi_vec] -> choose ksi_est_err 40/1(x)
  [phi_vec] -> choose ksi_est_err 39/1(x)
  Mux39/1 -> Interpreted MATLAB Function39/1
  cal abs 40/1(y) -> Mux39/1
  choose ksi_est_err 40/1(y) -> cal abs 40/1(x)
  [phi_squ_2_5] -> cal theta_phi agent 5/3(phi_squ_2_5)
  cal abs 39/1(y) -> Mux40/1
  Constant170/1 -> Mux39/2
  combine theta_err_ksi1/1(theta_phi_1_vec) -> [theta_phi_1_vec]
  [theta_phi_2_1] -> combine theta_err_ksi1/6(theta_phi_2_1)
  [theta_phi_1_4] -> combine theta_err_ksi1/4(theta_phi_1_4)
  [theta_phi_2_2] -> combine theta_err_ksi1/7(theta_phi_2_2)
  [theta_phi_1_2] -> combine theta_err_ksi1/2(theta_phi_1_2)
  [theta_phi_2_5] -> combine theta_err_ksi1/10(theta_phi_2_5)
  [theta_phi_2_4] -> combine theta_err_ksi1/9(theta_phi_2_4)
  combine theta_err_ksi1/2(theta_phi_2_vec) -> [theta_phi_2_vec]
  [theta_phi_1_1] -> combine theta_err_ksi1/1(theta_phi_1_1)
  [theta_phi_2_3] -> combine theta_err_ksi1/8(theta_phi_2_3)
  [theta_phi_1_5] -> combine theta_err_ksi1/5(theta_phi_1_5)
  [theta_phi_1_3] -> combine theta_err_ksi1/3(theta_phi_1_3)
  Constant172/1 -> cal ui agent 1/1(kai_u_1)
  Constant173/1 -> cal ui agent 1/2(kai_u_2)
  [theta_phi_1_vec] -> cal ui agent 1/4(theta_phi_1_vec)
  [theta_phi_2_vec] -> cal ui agent 1/5(theta_phi_2_vec)
  [dp_hat_vec] -> cal ui agent 1/6(dp_hat_vec)
  cal ui agent 1/1(ui_1) -> [ui_1]
  [dp_hat_vec] -> cal ui agent 2/6(dp_hat_vec)
  Constant175/1 -> cal ui agent 2/2(kai_u_2)
  [theta_phi_1_vec] -> cal ui agent 2/4(theta_phi_1_vec)
  Constant174/1 -> cal ui agent 2/1(kai_u_1)
  cal ui agent 2/1(ui_2) -> [ui_2]
  [theta_phi_2_vec] -> cal ui agent 2/5(theta_phi_2_vec)
  [d_chi_vec] -> cal ui agent 2/3(d_chi_vec)
  [d_chi_vec] -> cal ui agent 3/3(d_chi_vec)
  [theta_phi_1_vec] -> cal ui agent 3/4(theta_phi_1_vec)
  [theta_phi_2_vec] -> cal ui agent 3/5(theta_phi_2_vec)
  cal ui agent 3/1(ui_3) -> [ui_3]
  Constant177/1 -> cal ui agent 3/2(kai_u_2)
  [dp_hat_vec] -> cal ui agent 3/6(dp_hat_vec)
  Constant176/1 -> cal ui agent 3/1(kai_u_1)
  [dp_hat_vec] -> cal ui agent 4/6(dp_hat_vec)
  Constant178/1 -> cal ui agent 4/1(kai_u_1)
  Constant179/1 -> cal ui agent 4/2(kai_u_2)
  [theta_phi_2_vec] -> cal ui agent 4/5(theta_phi_2_vec)
  [d_chi_vec] -> cal ui agent 4/3(d_chi_vec)
  [theta_phi_1_vec] -> cal ui agent 4/4(theta_phi_1_vec)
  cal ui agent 4/1(ui_4) -> [ui_4]
  [d_chi_vec] -> cal ui agent 5/3(d_chi_vec)
  [theta_phi_1_vec] -> cal ui agent 5/4(theta_phi_1_vec)
  [theta_phi_2_vec] -> cal ui agent 5/5(theta_phi_2_vec)
  Constant181/1 -> cal ui agent 5/2(kai_u_2)
  [dp_hat_vec] -> cal ui agent 5/6(dp_hat_vec)
  Constant180/1 -> cal ui agent 5/1(kai_u_1)
  cal ui agent 5/1(ui_5) -> [ui_5]
  [ui_5] -> combine ui/5(ui_5)
  [ui_2] -> combine ui/2(ui_2)
  [ui_1] -> combine ui/1(ui_1)
  [ui_4] -> combine ui/4(ui_4)
  [ui_3] -> combine ui/3(ui_3)
  [dp_vec] -> cal disturbance observation error dp_tilt/1(dp_vec)
  [dp_hat_vec] -> cal disturbance observation error dp_tilt/2(dp_hat_vec)
  cal disturbance observation error dp_tilt/1(dp_tilt_vec) -> [dp_tilt_vec]
  [dp_hat_vec] -> To Workspace1/1
  [dp_vec] -> To Workspace2/1
  [dp_tilt_vec] -> To Workspace6/1
  Demux11/2 -> dp_tilt_1/2
  Demux11/1 -> dp_tilt_1/1
  Demux11/3 -> dp_tilt_1/3
  choose dp_tilt_1/1(y) -> Demux11/1
  [dp_tilt_vec] -> choose dp_tilt_5/1(x), choose dp_tilt_4/1(x), choose dp_tilt_3/1(x), choose dp_tilt_2/1(x), choose dp_tilt_1/1(x)
  Demux13/1 -> dp_tilt_2/1
  Demux13/2 -> dp_tilt_2/2
  Demux13/3 -> dp_tilt_2/3
  choose dp_tilt_2/1(y) -> Demux13/1
  Demux14/3 -> dp_tilt_3/3
  Demux14/1 -> dp_tilt_3/1
  choose dp_tilt_3/1(y) -> Demux14/1
  Demux14/2 -> dp_tilt_3/2
  Demux15/1 -> dp_tilt_4/1
  choose dp_tilt_4/1(y) -> Demux15/1
  Demux15/2 -> dp_tilt_4/2
  Demux15/3 -> dp_tilt_4/3
  choose dp_tilt_5/1(y) -> Demux16/1
  Demux16/3 -> dp_tilt_5/3
  Demux16/1 -> dp_tilt_5/1
  Demux16/2 -> dp_tilt_5/2
  Demux17/1 -> sigma_bar_v_tilt_1/1
  Demux17/2 -> sigma_bar_v_tilt_1/2
  choose sigma_bar_v_tilt_1/1(y) -> Demux17/1
  Demux19/2 -> sigma_bar_v_tilt_3/2
  Demux19/1 -> sigma_bar_v_tilt_3/1
  choose sigma_bar_v_tilt_3/1(y) -> Demux19/1
  Demux19/3 -> sigma_bar_v_tilt_3/3
  Demux17/3 -> sigma_bar_v_tilt_1/3
  choose sigma_bar_v_tilt_5/1(y) -> Demux21/1
  Demux21/2 -> sigma_bar_v_tilt_5/2
  [sigma_bar_v_tilt_vec] -> choose sigma_bar_v_tilt_5/1(x), choose sigma_bar_v_tilt_4/1(x), choose sigma_bar_v_tilt_3/1(x), choose sigma_bar_v_tilt_2/1(x), choose sigma_bar_v_tilt_1/1(x)
  Demux21/1 -> sigma_bar_v_tilt_5/1
  Demux21/3 -> sigma_bar_v_tilt_5/3
  choose sigma_bar_v_tilt_4/1(y) -> Demux20/1
  Demux20/3 -> sigma_bar_v_tilt_4/3
  Demux20/2 -> sigma_bar_v_tilt_4/2
  Demux18/3 -> sigma_bar_v_tilt_2/3
  Demux20/1 -> sigma_bar_v_tilt_4/1
  Demux18/1 -> sigma_bar_v_tilt_2/1
  choose sigma_bar_v_tilt_2/1(y) -> Demux18/1
  Demux18/2 -> sigma_bar_v_tilt_2/2
  Demux34/2 -> phi_2/2
  Demux36/1 -> phi_4/1
  Demux34/3 -> phi_2/3
  Demux36/2 -> phi_4/2
  Demux36/3 -> phi_4/3
  choose phi_4/1(y) -> Demux36/1
  Demux37/3 -> phi_5/3
  Demux37/1 -> phi_5/1
  Demux35/3 -> phi_3/3
  Demux35/1 -> phi_3/1
  Demux34/1 -> phi_2/1
  choose phi_2/1(y) -> Demux34/1
  Demux35/2 -> phi_3/2
  Demux33/2 -> phi_1/2
  choose phi_1/1(y) -> Demux33/1
  choose phi_3/1(y) -> Demux35/1
  Demux33/1 -> phi_1/1
  [phi_vec] -> choose phi_5/1(x), choose phi_4/1(x), choose phi_3/1(x), choose phi_2/1(x), choose phi_1/1(x)
  Demux33/3 -> phi_1/3
  choose phi_5/1(y) -> Demux37/1
  Demux37/2 -> phi_5/2
  [sigma_bar_v_hat_vec] -> To Workspace11/1
  [sigma_bar_v_vec] -> To Workspace12/1
  [sigma_bar_v_tilt_vec] -> To Workspace13/1
  Demux38/3 -> Mux43/1
  Mux41/1 -> compare err_eta_1 and chi_1/1
  Mux43/1 -> compare err_eta_1 and chi_1/3
  Demux39/2 -> Mux42/2
  Demux39/3 -> Mux43/2
  Demux39/1 -> Mux41/2
  Demux38/2 -> Mux42/1
  Mux42/1 -> compare err_eta_1 and chi_1/2
  Demux38/1 -> Mux41/1
  choose err_eta_1/1(y) -> Demux39/1
  [err_eta_vec] -> choose err_eta_1/1(x)
  [chi_vec] -> choose chi_1/1(x)
  choose chi_1/1(y) -> Demux38/1
  choose chi_2/1(y) -> Demux40/1
  [chi_vec] -> choose chi_2/1(x)
  [err_eta_vec] -> choose err_eta_2/1(x)
  Mux45/1 -> compare err_eta_2 and chi_2/2
  Demux40/2 -> Mux45/1
  Demux41/1 -> Mux44/2
  Demux41/2 -> Mux45/2
  Mux46/1 -> compare err_eta_2 and chi_2/3
  choose err_eta_2/1(y) -> Demux41/1
  Mux44/1 -> compare err_eta_2 and chi_2/1
  Demux40/1 -> Mux44/1
  Demux40/3 -> Mux46/1
  Demux41/3 -> Mux46/2
  Demux43/3 -> Mux49/2
  Demux42/3 -> Mux49/1
  choose err_eta_3/1(y) -> Demux43/1
  Mux47/1 -> compare err_eta_3 and chi_3/1
  Mux49/1 -> compare err_eta_3 and chi_3/3
  [err_eta_vec] -> choose err_eta_3/1(x)
  Demux42/1 -> Mux47/1
  Demux43/1 -> Mux47/2
  Demux43/2 -> Mux48/2
  [chi_vec] -> choose chi_3/1(x)
  Mux48/1 -> compare err_eta_3 and chi_3/2
  Demux42/2 -> Mux48/1
  choose chi_3/1(y) -> Demux42/1
  [chi_vec] -> choose chi_4/1(x)
  choose chi_4/1(y) -> Demux44/1
  Demux44/2 -> Mux51/1
  Demux44/1 -> Mux50/1
  Demux45/2 -> Mux51/2
  Demux45/3 -> Mux52/2
  Mux51/1 -> compare err_eta_4 and chi_4/2
  Mux50/1 -> compare err_eta_4 and chi_4/1
  Mux52/1 -> compare err_eta_4 and chi_4/3
  Demux45/1 -> Mux50/2
  choose err_eta_4/1(y) -> Demux45/1
  Demux44/3 -> Mux52/1
  [err_eta_vec] -> choose err_eta_4/1(x)
  Demux46/3 -> Mux55/1
  [err_eta_vec] -> choose err_eta_5/1(x)
  Mux55/1 -> compare err_eta_5 and chi_5/3
  choose err_eta_5/1(y) -> Demux47/1
  Mux53/1 -> compare err_eta_5 and chi_5/1
  Demux47/1 -> Mux53/2
  Demux47/2 -> Mux54/2
  Demux46/2 -> Mux54/1
  Demux46/1 -> Mux53/1
  [chi_vec] -> choose chi_5/1(x)
  choose chi_5/1(y) -> Demux46/1
  Mux54/1 -> compare err_eta_5 and chi_5/2
  Demux47/3 -> Mux55/2
  choose sigma_bar_v_hat_1/1(y) -> Demux48/1
  Demux57/3 -> Mux70/2
  choose sigma_bar_v_hat_5/1(y) -> Demux56/1
  [sigma_bar_v_hat_vec] -> choose sigma_bar_v_hat_5/1(x)
  Demux57/2 -> Mux69/2
  choose sigma_bar_v_5/1(y) -> Demux57/1
  Demux56/3 -> Mux70/1
  Demux56/2 -> Mux69/1
  Mux70/1 -> compare sigma_bar_v_5 and sigma_bar_v_hat_5/3
  [sigma_bar_v_vec] -> choose sigma_bar_v_1/1(x)
  Mux57/1 -> compare sigma_bar_v_1 and sigma_bar_v_hat_1/2
  Demux49/3 -> Mux58/2
  Demux49/2 -> Mux57/2
  Demux48/3 -> Mux58/1
  Demux57/1 -> Mux68/2
  [sigma_bar_v_vec] -> choose sigma_bar_v_4/1(x)
  Demux56/1 -> Mux68/1
  [sigma_bar_v_hat_vec] -> choose sigma_bar_v_hat_1/1(x)
  Mux67/1 -> compare sigma_bar_v_4 and sigma_bar_v_hat_4/3
  Demux49/1 -> Mux56/2
  choose sigma_bar_v_4/1(y) -> Demux55/1
  Mux66/1 -> compare sigma_bar_v_4 and sigma_bar_v_hat_4/2
  Demux55/2 -> Mux66/2
  Demux54/2 -> Mux66/1
  Demux54/1 -> Mux65/1
  [sigma_bar_v_hat_vec] -> choose sigma_bar_v_hat_4/1(x)
  [sigma_bar_v_hat_vec] -> choose sigma_bar_v_hat_3/1(x)
  Demux54/3 -> Mux67/1
  Mux63/1 -> compare sigma_bar_v_3 and sigma_bar_v_hat_3/2
  [sigma_bar_v_vec] -> choose sigma_bar_v_5/1(x)
  Demux52/1 -> Mux62/1
  [sigma_bar_v_vec] -> choose sigma_bar_v_3/1(x)
  Demux53/2 -> Mux63/2
  Demux53/3 -> Mux64/2
  Mux65/1 -> compare sigma_bar_v_4 and sigma_bar_v_hat_4/1
  Mux62/1 -> compare sigma_bar_v_3 and sigma_bar_v_hat_3/1
  Mux64/1 -> compare sigma_bar_v_3 and sigma_bar_v_hat_3/3
  Demux52/3 -> Mux64/1
  Demux55/3 -> Mux67/2
  Mux56/1 -> compare sigma_bar_v_1 and sigma_bar_v_hat_1/1
  Demux51/3 -> Mux61/2
  Demux52/2 -> Mux63/1
  Demux50/3 -> Mux61/1
  choose sigma_bar_v_2/1(y) -> Demux51/1
  Demux48/2 -> Mux57/1
  Demux55/1 -> Mux65/2
  Mux59/1 -> compare sigma_bar_v_2 and sigma_bar_v_hat_2/1
  Mux61/1 -> compare sigma_bar_v_2 and sigma_bar_v_hat_2/3
  [sigma_bar_v_vec] -> choose sigma_bar_v_2/1(x)
  Mux68/1 -> compare sigma_bar_v_5 and sigma_bar_v_hat_5/1
  choose sigma_bar_v_1/1(y) -> Demux49/1
  Demux53/1 -> Mux62/2
  Demux50/1 -> Mux59/1
  Mux58/1 -> compare sigma_bar_v_1 and sigma_bar_v_hat_1/3
  Demux51/1 -> Mux59/2
  choose sigma_bar_v_hat_3/1(y) -> Demux52/1
  Mux69/1 -> compare sigma_bar_v_5 and sigma_bar_v_hat_5/2
  Demux51/2 -> Mux60/2
  choose sigma_bar_v_hat_4/1(y) -> Demux54/1
  Demux48/1 -> Mux56/1
  [sigma_bar_v_hat_vec] -> choose sigma_bar_v_hat_2/1(x)
  Mux60/1 -> compare sigma_bar_v_2 and sigma_bar_v_hat_2/2
  Demux50/2 -> Mux60/1
  choose sigma_bar_v_hat_2/1(y) -> Demux50/1
  choose sigma_bar_v_3/1(y) -> Demux53/1
  choose dp_1/1(y) -> Demux59/1
  Demux61/1 -> Mux74/2
  Mux83/1 -> compare dp_5 and dp_hat_5/1
  Demux58/2 -> Mux72/1
  [dp_vec] -> choose dp_2/1(x)
  Mux76/1 -> compare dp_2 and dp_hat_2/3
  Mux71/1 -> compare dp_1 and dp_hat_1/1
  Demux62/3 -> Mux79/1
  Mux79/1 -> compare dp_3 and dp_hat_3/3
  Demux61/3 -> Mux76/2
  Demux62/2 -> Mux78/1
  Mux77/1 -> compare dp_3 and dp_hat_3/1
  Demux65/3 -> Mux82/2
  [dp_vec] -> choose dp_3/1(x)
  Mux80/1 -> compare dp_4 and dp_hat_4/1
  Demux60/3 -> Mux76/1
  Mux73/1 -> compare dp_1 and dp_hat_1/3
  Demux63/1 -> Mux77/2
  Demux63/3 -> Mux79/2
  Demux63/2 -> Mux78/2
  Demux64/3 -> Mux82/1
  Demux62/1 -> Mux77/1
  Mux78/1 -> compare dp_3 and dp_hat_3/2
  [dp_vec] -> choose dp_5/1(x)
  [dp_hat_vec] -> choose dp_hat_3/1(x)
  [dp_hat_vec] -> choose dp_hat_4/1(x)
  Demux64/1 -> Mux80/1
  Demux64/2 -> Mux81/1
  Demux65/2 -> Mux81/2
  Demux65/1 -> Mux80/2
  Demux59/1 -> Mux71/2
  Demux60/1 -> Mux74/1
  choose dp_4/1(y) -> Demux65/1
  Mux81/1 -> compare dp_4 and dp_hat_4/2
  Demux67/1 -> Mux83/2
  choose dp_2/1(y) -> Demux61/1
  [dp_hat_vec] -> choose dp_hat_1/1(x)
  Demux59/2 -> Mux72/2
  [dp_vec] -> choose dp_4/1(x)
  choose dp_hat_3/1(y) -> Demux62/1
  Mux82/1 -> compare dp_4 and dp_hat_4/3
  Mux72/1 -> compare dp_1 and dp_hat_1/2
  Demux59/3 -> Mux73/2
  [dp_vec] -> choose dp_1/1(x)
  Mux74/1 -> compare dp_2 and dp_hat_2/1
  Mux85/1 -> compare dp_5 and dp_hat_5/3
  Demux66/3 -> Mux85/1
  choose dp_5/1(y) -> Demux67/1
  Demux66/2 -> Mux84/1
  choose dp_hat_1/1(y) -> Demux58/1
  choose dp_hat_5/1(y) -> Demux66/1
  Mux84/1 -> compare dp_5 and dp_hat_5/2
  choose dp_3/1(y) -> Demux63/1
  Demux67/3 -> Mux85/2
  Demux66/1 -> Mux83/1
  Demux61/2 -> Mux75/2
  choose dp_hat_2/1(y) -> Demux60/1
  Mux75/1 -> compare dp_2 and dp_hat_2/2
  Demux58/1 -> Mux71/1
  [dp_hat_vec] -> choose dp_hat_2/1(x)
  Demux67/2 -> Mux84/2
  Demux60/2 -> Mux75/1
  choose dp_hat_4/1(y) -> Demux64/1
  [dp_hat_vec] -> choose dp_hat_5/1(x)
  Demux58/3 -> Mux73/1
  [phi_vec] -> To Workspace16/1
  [chi_vec] -> To Workspace15/1
  Constant280/1 -> Mux129/3
  Mux128/1 -> Interpreted MATLAB Function50/1
  choose eta_est_err_tilt 13/1(y) -> cal abs 45/1(x)
  choose eta_est_err_tilt 12/1(y) -> cal abs 44/1(x)
  [ksi_est_err_tilt_vec] -> choose eta_est_err_tilt 14/1(x)
  cal abs 48/1(y) -> Mux124/1
  trans to column46/1(y) -> [ksi_est_err_squ_2_node_3], Display80/1
  [eta_est_err_tilt_vec] -> choose eta_est_err_tilt 10/1(x)
  Constant247/1 -> Mux109/2
  [ksi0] -> cal lumped observation error agent 2/4(ksi0)
  [theta_eta_est_err_tilt_1_vec] -> fixed-time distributed follower desire velocity observer agent 2/3(theta_eta_est_err_tilt_1_vec)
  Interpreted MATLAB Function47/1 -> trans to column47/1(x)
  Constant273/1 -> Mux123/3
  Constant227/1 -> cal lumped observation error agent 2/1(wij)
  Interpreted MATLAB Function46/1 -> trans to column46/1(x)
  choose eta_est_err_tilt 15/1(y) -> cal abs 47/1(x)
  choose eta_est_err_tilt 5/1(y) -> cal abs 56/1(x)
  choose eta_est_err_tilt 14/1(y) -> cal abs 46/1(x)
  cal abs 43/1(y) -> Mux126/1
  Constant218/1 -> Mux120/3
  choose eta_est_err_tilt 16/1(y) -> cal abs 48/1(x)
  Constant220/1 -> Mux122/2
  trans to column45/1(y) -> [ksi_est_err_squ_1_node_1], Display84/1
  Constant200/1 -> fixed-time distributed follower desire velocity observer agent 1/1(l1v)
  Constant281/1 -> Mux128/2
  Constant214/1 -> Add4/2
  Interpreted MATLAB Function50/1 -> trans to column50/1(x)
  Add3/1 -> Demux76/1
  trans to column50/1(y) -> [ksi_est_err_squ_2_node_5], Display85/1
  cal theta_ksi_est_err_tilt agent 1/1(theta_ksi_est_err_tilt_1_1) -> [theta_ksi_est_err_tilt_1_1]
  [eta_est_err_squ_1_node_3] -> cal theta_eta_est_err_tilt agent 3/2(eta_est_err_squ_1_node_3)
  Add8/1 -> Demux97/1
  [eta_est_err_squ_1_node_2] -> cal theta_eta_est_err_tilt agent 2/2(eta_est_err_squ_1_node_2)
  Constant263/1 -> fixed-time distributed follower desire position observer agent 3/1(l1p)
  Mux134/1 -> ksi_d_est_3/2
  cal theta_ksi_est_err_tilt agent 5/2(theta_ksi_est_err_tilt_2_5) -> [theta_ksi_est_err_tilt_2_5]
  [eta_d_est_vec] -> fixed-time distributed follower desire position observer agent 1/3(eta_d_est_vec)
  Interpreted MATLAB Function56/1 -> trans to column56/1(x)
  cal theta_ksi_est_err_tilt agent 2/2(theta_ksi_est_err_tilt_2_2) -> [theta_ksi_est_err_tilt_2_2]
  Constant248/1 -> Mux109/3
  Constant252/1 -> fixed-time distributed follower desire position observer agent 3/2(l2p)
  Mux135/1 -> ksi_d_est_3/3
  trans to column48/1(y) -> [ksi_est_err_squ_2_node_4], Display82/1
  Demux93/2 -> Mux130/2
  [theta_eta_est_err_tilt_2_3] -> combine lumped follower velocity observation error/8(theta_eta_est_err_tilt_2_3)
  [theta_eta_est_err_tilt_1_3] -> combine lumped follower velocity observation error/3(theta_eta_est_err_tilt_1_3)
  position observe Integrator 2/1 -> [ksi_d_est_2], Demux92/1
  Demux95/3 -> Mux135/2
  [ksi0] -> cal lumped observation error agent 1/4(ksi0)
  Demux94/2 -> Mux134/1
  [theta_eta_est_err_tilt_2_vec] -> fixed-time distributed follower desire velocity observer agent 5/4(theta_eta_est_err_tilt_2_vec)
  Mux109/1 -> Interpreted MATLAB Function41/1
  [ksi0] -> Add6/1
  velocity observe Integrator 5/1 -> [eta_d_est_5], Demux77/1
  Constant268/1 -> Mux121/2
  Demux93/1 -> Mux119/2
  fixed-time distributed follower desire position observer agent 2/1(d_ksi_d_est_2) -> position observe Integrator 2/1
  Demux93/3 -> Mux132/2
  [theta_ksi_est_err_tilt_1_vec] -> fixed-time distributed follower desire position observer agent 3/4(theta_ksi_est_err_tilt_1_vec)
  [ksi_est_err_squ_1_node_3] -> cal theta_ksi_est_err_tilt agent 3/2(ksi_est_err_squ_1_node_3)
  Constant216/1 -> Mux126/3
  Mux108/1 -> ksi_d_est_1/3
  trans to column43/1(y) -> [ksi_est_err_squ_2_node_2], Display78/1
  Mux113/1 -> Interpreted MATLAB Function56/1
  [ksi_est_err_tilt_vec] -> choose eta_est_err_tilt 18/1(x)
  Add6/1 -> Demux93/1
  Mux119/1 -> ksi_d_est_2/1
  [theta_eta_est_err_tilt_1_1] -> combine lumped follower velocity observation error/1(theta_eta_est_err_tilt_1_1)
  Interpreted MATLAB Function53/1 -> trans to column53/1(x)
  cal theta_eta_est_err_tilt agent 3/1(theta_eta_est_err_tilt_1_3) -> [theta_eta_est_err_tilt_1_3]
  Demux88/3 -> Mux108/2
  Demux88/1 -> Mux86/2
  Add5/1 -> Demux88/1
  [eta_est_err_tilt_3] -> "combine lumped follower observation error "/8(eta_est_err_tilt_3)
  Constant261/1 -> Mux114/3
  Constant270/1 -> Mux124/2
  Demux73/2 -> Mux100/1
  Constant267/1 -> Mux122/3
  cal abs 60/1(y) -> Mux118/1
  [theta_ksi_est_err_tilt_1_3] -> combine lumped follower position observation error/3(theta_ksi_est_err_tilt_1_3)
  [theta_ksi_est_err_tilt_2_4] -> combine lumped follower position observation error/9(theta_ksi_est_err_tilt_2_4)
  Mux117/1 -> Interpreted MATLAB Function59/1
  cal theta_ksi_est_err_tilt agent 4/2(theta_ksi_est_err_tilt_2_4) -> [theta_ksi_est_err_tilt_2_4]
  trans to column47/1(y) -> [ksi_est_err_squ_1_node_3], Display81/1
  Add1/1 -> Demux72/1
  [ksi0] -> cal lumped observation error agent 3/4(ksi0)
  Constant203/1 -> fixed-time distributed follower desire velocity observer agent 2/1(l1v)
  cal abs 44/1(y) -> Mux128/1
  [eta_d_est_vec] -> cal lumped observation error agent 1/6(eta_d_est_vec)
  Mux127/1 -> Interpreted MATLAB Function49/1
  Constant278/1 -> Mux125/3
  [theta_eta_est_err_tilt_1_vec] -> fixed-time distributed follower desire velocity observer agent 5/3(theta_eta_est_err_tilt_1_vec)
  [ksi_est_err_tilt_4] -> "combine lumped follower observation error "/4(ksi_est_err_tilt_4)
  [ksi_est_err_tilt_vec] -> choose eta_est_err_tilt 12/1(x)
  trans to column51/1(y) -> [ksi_est_err_squ_1_node_5], Display86/1
  Interpreted MATLAB Function51/1 -> trans to column51/1(x)
  trans to column56/1(y) -> [eta_est_err_squ_1_node_3], Display90/1
  choose eta_est_err_tilt 18/1(y) -> cal abs 50/1(x)
  [ksi_est_err_tilt_vec] -> cal theta_ksi_est_err_tilt agent 1/4(ksi_est_err_tilt_vec)
  Mux103/1 -> eta_d_est_4/2
  velocity observe Integrator 4/1 -> [eta_d_est_4], Demux75/1
  Demux77/2 -> Mux106/1
  Demux77/1 -> Mux105/1
  Mux107/1 -> eta_d_est_5/3
  fixed-time distributed follower desire velocity observer agent 5/1(d_eta_d_est_5) -> velocity observe Integrator 5/1
  [theta_eta_est_err_tilt_2_5] -> combine lumped follower velocity observation error/10(theta_eta_est_err_tilt_2_5)
  Mux104/1 -> eta_d_est_4/3
  Demux74/3 -> Mux101/2
  Constant205/1 -> fixed-time distributed follower desire velocity observer agent 3/2(l2v)
  fixed-time distributed follower desire velocity observer agent 3/1(d_eta_d_est_3) -> velocity observe Integrator 3/1
  Demux74/2 -> Mux100/2
  Demux75/2 -> Mux103/1
  Constant207/1 -> Add2/2
  Demux76/3 -> Mux104/2
  Demux75/3 -> Mux104/1
  cal lumped observation error agent 4/2(eta_est_err_tilt_4) -> [eta_est_err_tilt_4]
  Mux95/1 -> eta_d_est_2/1
  velocity observe Integrator 3/1 -> [eta_d_est_3], Demux73/1
  velocity observe Integrator 2/1 -> [eta_d_est_2], Demux71/1
  Demux72/1 -> Mux95/2
  [eta0] -> Add2/1
  [eta_est_err_tilt_5] -> "combine lumped follower observation error "/10(eta_est_err_tilt_5)
  cal abs 45/1(y) -> Mux120/1
  Add/1 -> Demux70/1
  cal lumped observation error agent 2/1(ksi_est_err_tilt_2) -> [ksi_est_err_tilt_2]
  cal theta_eta_est_err_tilt agent 5/2(theta_eta_est_err_tilt_2_5) -> [theta_eta_est_err_tilt_2_5]
  fixed-time distributed follower desire velocity observer agent 2/1(d_eta_d_est_2) -> velocity observe Integrator 2/1
  [theta_eta_est_err_tilt_2_vec] -> fixed-time distributed follower desire velocity observer agent 2/4(theta_eta_est_err_tilt_2_vec)
  Mux98/1 -> eta_d_est_2/3
  [eta_est_err_tilt_vec] -> cal theta_eta_est_err_tilt agent 4/4(eta_est_err_tilt_vec)
  [eta_d_est_5] -> combine follower desire velocity estimaters/5(eta_d_est_5)
  trans to column60/1(y) -> [eta_est_err_squ_1_node_5], Display95/1
  cal lumped observation error agent 3/1(ksi_est_err_tilt_3) -> [ksi_est_err_tilt_3]
  [eta_est_err_squ_2_node_2] -> cal theta_eta_est_err_tilt agent 2/3(eta_est_err_squ_2_node_2)
  cal theta_eta_est_err_tilt agent 3/2(theta_eta_est_err_tilt_2_3) -> [theta_eta_est_err_tilt_2_3]
  cal theta_eta_est_err_tilt agent 1/2(theta_eta_est_err_tilt_2_1) -> [theta_eta_est_err_tilt_2_1]
  [eta_est_err_tilt_vec] -> cal theta_eta_est_err_tilt agent 2/4(eta_est_err_tilt_vec)
  [eta_est_err_squ_1_node_4] -> cal theta_eta_est_err_tilt agent 4/2(eta_est_err_squ_1_node_4)
  cal theta_eta_est_err_tilt agent 2/2(theta_eta_est_err_tilt_2_2) -> [theta_eta_est_err_tilt_2_2]
  [eta_est_err_tilt_vec] -> choose eta_est_err_tilt 9/1(x)
  Demux72/2 -> Mux96/2
  [theta_eta_est_err_tilt_2_1] -> combine lumped follower velocity observation error/6(theta_eta_est_err_tilt_2_1)
  [eta_est_err_tilt_vec] -> choose eta_est_err_tilt 5/1(x)
  [eta_est_err_tilt_vec] -> cal theta_eta_est_err_tilt agent 1/4(eta_est_err_tilt_vec)
  choose eta_est_err_tilt 10/1(y) -> cal abs 42/1(x)
  [eta_est_err_squ_1_node_1] -> cal theta_eta_est_err_tilt agent 1/2(eta_est_err_squ_1_node_1)
  [theta_eta_est_err_tilt_1_4] -> combine lumped follower velocity observation error/4(theta_eta_est_err_tilt_1_4)
  [theta_ksi_est_err_tilt_2_5] -> combine lumped follower position observation error/10(theta_ksi_est_err_tilt_2_5)
  Constant259/1 -> Mux116/3
  choose eta_est_err_tilt 4/1(y) -> cal abs 55/1(x)
  choose eta_est_err_tilt 8/1(y) -> cal abs 59/1(x)
  Mux118/1 -> Interpreted MATLAB Function60/1
  Constant266/1 -> Mux117/3
  Constant262/1 -> Mux118/2
  Constant255/1 -> Mux113/3
  [eta_est_err_tilt_vec] -> choose eta_est_err_tilt 7/1(x)
  [ksi_d_est_vec] -> cal lumped observation error agent 5/3(ksi_d_est_vec)
  Interpreted MATLAB Function58/1 -> trans to column58/1(x)
  [eta_d_est_2] -> combine follower desire velocity estimaters/2(eta_d_est_2)
  Mux114/1 -> Interpreted MATLAB Function57/1
  cal abs 59/1(y) -> Mux114/1
  Constant260/1 -> Mux114/2
  Interpreted MATLAB Function55/1 -> trans to column55/1(x)
  trans to column58/1(y) -> [eta_est_err_squ_1_node_4], Display92/1
  Constant228/1 -> cal lumped observation error agent 2/2(w0)
  [theta_ksi_est_err_tilt_2_1] -> combine lumped follower position observation error/6(theta_ksi_est_err_tilt_2_1)
  Constant249/1 -> Mux111/2
  Constant265/1 -> Mux117/2
  cal abs 51/1(y) -> Mux125/1
  Mux112/1 -> Interpreted MATLAB Function55/1
  Mux111/1 -> Interpreted MATLAB Function53/1
  Constant250/1 -> Mux111/3
  cal theta_eta_est_err_tilt agent 5/1(theta_eta_est_err_tilt_1_5) -> [theta_eta_est_err_tilt_1_5]
  choose eta_est_err_tilt 3/1(y) -> cal abs 54/1(x)
  trans to column52/1(y) -> [eta_est_err_squ_2_node_2], Display87/1
  [ksi_est_err_tilt_2] -> "combine lumped follower observation error "/2(ksi_est_err_tilt_2)
  cal abs 42/1(y) -> Mux117/1
  Constant254/1 -> Mux113/2
  Constant256/1 -> Mux112/2
  [ksi_est_err_tilt_5] -> "combine lumped follower observation error "/5(ksi_est_err_tilt_5)
  Demux76/1 -> Mux102/2
  [theta_eta_est_err_tilt_1_5] -> combine lumped follower velocity observation error/5(theta_eta_est_err_tilt_1_5)
  choose eta_est_err_tilt 1/1(y) -> cal abs 41/1(x)
  choose eta_est_err_tilt 9/1(y) -> cal abs 60/1(x)
  Mux110/1 -> Interpreted MATLAB Function52/1
  Constant251/1 -> Mux110/2
  Mux124/1 -> Interpreted MATLAB Function47/1
  cal lumped observation error agent 5/1(ksi_est_err_tilt_5) -> [ksi_est_err_tilt_5]
  [eta_est_err_tilt_2] -> "combine lumped follower observation error "/7(eta_est_err_tilt_2)
  Mux123/1 -> Interpreted MATLAB Function46/1
  [ksi_d_est_vec] -> cal lumped observation error agent 3/3(ksi_d_est_vec)
  Constant242/1 -> cal lumped observation error agent 5/2(w0)
  [ksi_d_est_vec] -> cal lumped observation error agent 4/3(ksi_d_est_vec)
  Mux105/1 -> eta_d_est_5/1
  [ksi_est_err_squ_2_node_1] -> cal theta_ksi_est_err_tilt agent 1/3(ksi_est_err_squ_2_node_1)
  [eta_est_err_tilt_4] -> "combine lumped follower observation error "/9(eta_est_err_tilt_4)
  Add7/1 -> Demux95/1
  Constant217/1 -> Mux120/2
  Constant236/1 -> cal lumped observation error agent 4/1(wij)
  [eta0] -> cal lumped observation error agent 1/7(eta0)
  [eta0] -> cal lumped observation error agent 2/7(eta0)
  choose eta_est_err_tilt 17/1(y) -> cal abs 49/1(x)
  cal lumped observation error agent 1/2(eta_est_err_tilt_1) -> [eta_est_err_tilt_1]
  Demux77/3 -> Mux107/1
  cal lumped observation error agent 1/1(ksi_est_err_tilt_1) -> [ksi_est_err_tilt_1]
  trans to column44/1(y) -> [ksi_est_err_squ_1_node_2], Display79/1
  [eta_d_est_vec] -> cal lumped observation error agent 2/6(eta_d_est_vec)
  cal lumped observation error agent 4/1(ksi_est_err_tilt_4) -> [ksi_est_err_tilt_4]
  Mux93/1 -> eta_d_est_1/2
  Constant199/1 -> fixed-time distributed follower desire velocity observer agent 1/2(l2v)
  Demux69/2 -> Mux93/1
  Mux100/1 -> eta_d_est_3/2
  Mux94/1 -> eta_d_est_1/3
  Demux73/1 -> Mux99/1
  [ksi_d_est_3] -> combine leader position estimaters/3(ksi_d_est_3)
  Demux70/2 -> Mux93/2
  [eta0] -> Add/1
  [ksi0] -> cal position estimate error/2(ksi0)
  Demux69/3 -> Mux94/1
  fixed-time distributed follower desire position observer agent 3/1(d_ksi_d_est_3) -> position observe Integrator 3/1
  cal theta_eta_est_err_tilt agent 4/2(theta_eta_est_err_tilt_2_4) -> [theta_eta_est_err_tilt_2_4]
  [eta_d_est_4] -> combine follower desire velocity estimaters/4(eta_d_est_4)
  [eta_d_est_1] -> combine follower desire velocity estimaters/1(eta_d_est_1)
  Constant233/1 -> cal lumped observation error agent 3/2(w0)
  choose eta_est_err_tilt 20/1(y) -> cal abs 53/1(x)
  Demux78/1 -> Mux86/1
  Constant215/1 -> Mux126/2
  Demux86/3 -> eta_est_err_1/3
  Demux89/2 -> eta_est_err_3/2
  Demux87/1 -> eta_est_err_2/1
  Constant275/1 -> Mux127/2
  trans to column57/1(y) -> [eta_est_err_squ_2_node_4], Display91/1
  [ksi_est_err_squ_1_node_5] -> cal theta_ksi_est_err_tilt agent 5/2(ksi_est_err_squ_1_node_5)
  Interpreted MATLAB Function57/1 -> trans to column57/1(x)
  divide eta_est_err/2(eta_est_err_2) -> Demux87/1
  [ksi_est_err_squ_1_node_2] -> cal theta_ksi_est_err_tilt agent 2/2(ksi_est_err_squ_1_node_2)
  Demux85/2 -> ksi_est_err_5/2
  Demux90/1 -> eta_est_err_4/1
  trans to column49/1(y) -> [ksi_est_err_squ_1_node_4], Display83/1
  cal theta_ksi_est_err_tilt agent 3/1(theta_ksi_est_err_tilt_1_3) -> [theta_ksi_est_err_tilt_1_3]
  cal abs 49/1(y) -> Mux123/1
  Demux90/2 -> eta_est_err_4/2
  choose eta_est_err_tilt 7/1(y) -> cal abs 58/1(x)
  Mux86/1 -> ksi_d_est_1/1
  Constant282/1 -> Mux128/3
  [eta_est_err_squ_2_node_4] -> cal theta_eta_est_err_tilt agent 4/3(eta_est_err_squ_2_node_4)
  Mux130/1 -> ksi_d_est_2/2
  Interpreted MATLAB Function60/1 -> trans to column60/1(x)
  Constant190/1 -> fixed-time distributed follower desire position observer agent 5/1(l1p)
  cal theta_eta_est_err_tilt agent 1/1(theta_eta_est_err_tilt_1_1) -> [theta_eta_est_err_tilt_1_1]
  Demux87/2 -> eta_est_err_2/2
  Mux131/1 -> ksi_d_est_5/3
  fixed-time distributed follower desire position observer agent 1/1(d_ksi_d_est_1) -> position observe Integrator 1/1
  Demux84/1 -> ksi_est_err_4/1
  cal theta_ksi_est_err_tilt agent 3/2(theta_ksi_est_err_tilt_2_3) -> [theta_ksi_est_err_tilt_2_3]
  Constant201/1 -> Add/2
  divide eta_est_err/4(eta_est_err_4) -> Demux90/1
  Constant197/1 -> fixed-time distributed follower desire position observer agent 1/1(l1p)
  Constant202/1 -> fixed-time distributed follower desire velocity observer agent 2/2(l2v)
  position observe Integrator 5/1 -> [ksi_d_est_5], Demux68/1
  Demux85/3 -> ksi_est_err_5/3
  Constant224/1 -> cal lumped observation error agent 1/2(w0)
  Demux85/1 -> ksi_est_err_5/1
  cal abs 50/1(y) -> Mux127/1
  Mux97/1 -> ksi_d_est_1/2
  [eta_est_err_tilt_vec] -> choose eta_est_err_tilt 2/1(x)
  cal abs 58/1(y) -> Mux116/1
  Demux84/2 -> ksi_est_err_4/2
  [eta_est_err_tilt_vec] -> choose eta_est_err_tilt 8/1(x)
  Demux94/3 -> Mux135/1
  divide ksi_est_err/4(ksi_est_err_4) -> Demux84/1
  Mux89/1 -> ksi_d_est_4/3
  Demux82/3 -> ksi_est_err_2/3
  Mux120/1 -> Interpreted MATLAB Function42/1
  [ksi_est_err_tilt_vec] -> choose eta_est_err_tilt 16/1(x)
  cal abs 47/1(y) -> Mux121/1
  Demux92/2 -> Mux130/1
  Constant240/1 -> cal lumped observation error agent 5/1(wij)
  [eta0] -> Add3/1
  Demux83/3 -> ksi_est_err_3/3
  Constant213/1 -> fixed-time distributed follower desire velocity observer agent 5/1(l1v)
  [theta_ksi_est_err_tilt_1_4] -> combine lumped follower position observation error/4(theta_ksi_est_err_tilt_1_4)
  Demux86/2 -> eta_est_err_1/2
  Demux88/2 -> Mux97/2
  Demux81/1 -> ksi_est_err_1/1
  [theta_ksi_est_err_tilt_1_2] -> combine lumped follower position observation error/2(theta_ksi_est_err_tilt_1_2)
  Demux82/2 -> ksi_est_err_2/2
  [ksi_d_est_5] -> combine leader position estimaters/5(ksi_d_est_5)
  divide ksi_est_err/2(ksi_est_err_2) -> Demux82/1
  Demux91/1 -> eta_est_err_5/1
  Constant211/1 -> Add3/2
  position observe Integrator 3/1 -> [ksi_d_est_3], Demux94/1
  cal theta_ksi_est_err_tilt agent 2/1(theta_ksi_est_err_tilt_1_2) -> [theta_ksi_est_err_tilt_1_2]
  [eta_est_err_squ_1_node_5] -> cal theta_eta_est_err_tilt agent 5/2(eta_est_err_squ_1_node_5)
  divide ksi_est_err/1(ksi_est_err_1) -> Demux81/1
  cal theta_ksi_est_err_tilt agent 5/1(theta_ksi_est_err_tilt_1_5) -> [theta_ksi_est_err_tilt_1_5]
  [theta_ksi_est_err_tilt_1_vec] -> fixed-time distributed follower desire position observer agent 2/4(theta_ksi_est_err_tilt_1_vec)
  Constant246/1 -> Mux115/3
  cal abs 53/1(y) -> Mux129/1
  [theta_ksi_est_err_tilt_2_vec] -> fixed-time distributed follower desire position observer agent 1/5(theta_ksi_est_err_tilt_2_vec)
  Demux82/1 -> ksi_est_err_2/1
  trans to column55/1(y) -> [eta_est_err_squ_2_node_3], Display89/1
  [eta_d_est_vec] -> fixed-time distributed follower desire position observer agent 4/3(eta_d_est_vec)
  Demux68/3 -> Mux131/1
  [ksi_est_err_tilt_vec] -> cal theta_ksi_est_err_tilt agent 3/4(ksi_est_err_tilt_vec)
  Interpreted MATLAB Function44/1 -> trans to column44/1(x)
  fixed-time distributed follower desire position observer agent 5/1(d_ksi_d_est_5) -> position observe Integrator 5/1
  [theta_ksi_est_err_tilt_2_vec] -> fixed-time distributed follower desire position observer agent 2/5(theta_ksi_est_err_tilt_2_vec)
  Demux78/2 -> Mux97/1
  Constant189/1 -> fixed-time distributed follower desire position observer agent 5/2(l2p)
  [theta_ksi_est_err_tilt_2_vec] -> fixed-time distributed follower desire position observer agent 5/5(theta_ksi_est_err_tilt_2_vec)
  Interpreted MATLAB Function49/1 -> trans to column49/1(x)
  cal abs 56/1(y) -> Mux113/1
  trans to column59/1(y) -> [eta_est_err_squ_2_node_5], Display94/1
  [eta0] -> cal lumped observation error agent 5/7(eta0)
  Demux78/3 -> Mux108/1
  [ksi_est_err_squ_2_node_3] -> cal theta_ksi_est_err_tilt agent 3/3(ksi_est_err_squ_2_node_3)
  [eta_est_err_tilt_vec] -> cal theta_eta_est_err_tilt agent 3/4(eta_est_err_tilt_vec)
  Constant206/1 -> fixed-time distributed follower desire velocity observer agent 3/1(l1v)
  [eta_d_est_3] -> combine follower desire velocity estimaters/3(eta_d_est_3)
  Constant192/1 -> Add9/2
  [eta0] -> cal velocity estimate error/2(eta0)
  Mux91/1 -> ksi_d_est_5/2
  Demux71/2 -> Mux96/1
  Interpreted MATLAB Function45/1 -> trans to column45/1(x)
  [eta_d_est_vec] -> cal lumped observation error agent 5/6(eta_d_est_vec)
  [ksi0] -> Add7/1
  [ksi_est_err_squ_1_node_1] -> cal theta_ksi_est_err_tilt agent 1/2(ksi_est_err_squ_1_node_1)
  [ksi0] -> Add9/1
  [ksi_est_err_tilt_1] -> "combine lumped follower observation error "/1(ksi_est_err_tilt_1)
  [eta_d_est_vec] -> fixed-time distributed follower desire position observer agent 3/3(eta_d_est_vec)
  [eta_d_est_vec] -> fixed-time distributed follower desire position observer agent 5/3(eta_d_est_vec)
  fixed-time distributed follower desire velocity observer agent 4/1(d_eta_d_est_4) -> velocity observe Integrator 4/1
  Mux90/1 -> ksi_d_est_5/1
  Constant272/1 -> Mux123/2
  Constant223/1 -> cal lumped observation error agent 1/1(wij)
  [eta0] -> cal lumped observation error agent 3/7(eta0)
  [eta_est_err_squ_2_node_5] -> cal theta_eta_est_err_tilt agent 5/3(eta_est_err_squ_2_node_5)
  Demux80/1 -> Mux90/2
  Constant187/1 -> fixed-time distributed follower desire position observer agent 4/1(l1p)
  Mux88/1 -> ksi_d_est_4/2
  Constant209/1 -> fixed-time distributed follower desire velocity observer agent 4/2(l2v)
  Add4/1 -> Demux79/1
  Constant232/1 -> cal lumped observation error agent 3/1(wij)
  [ksi_est_err_tilt_vec] -> choose eta_est_err_tilt 13/1(x)
  Mux87/1 -> ksi_d_est_4/1
  position observe Integrator 1/1 -> [ksi_d_est_1], Demux78/1
  Demux80/3 -> Mux131/2
  [ksi0] -> cal lumped observation error agent 5/4(ksi0)
  [ksi_d_est_vec] -> cal position estimate error/1(ksi_d_est_vec)
  choose eta_est_err_tilt 6/1(y) -> cal abs 57/1(x)
  Demux73/3 -> Mux101/1
  Demux69/1 -> Mux92/1
  Constant204/1 -> Add1/2
  [theta_ksi_est_err_tilt_1_5] -> combine lumped follower position observation error/5(theta_ksi_est_err_tilt_1_5)
  Demux96/2 -> Mux88/1
  [ksi_est_err_tilt_vec] -> choose eta_est_err_tilt 19/1(x)
  position observe Integrator 4/1 -> [ksi_d_est_4], Demux96/1
  Demux72/3 -> Mux98/2
  Constant274/1 -> Add7/2
  cal theta_eta_est_err_tilt agent 2/1(theta_eta_est_err_tilt_1_2) -> [theta_eta_est_err_tilt_1_2]
  Demux74/1 -> Mux99/2
  cal theta_ksi_est_err_tilt agent 4/1(theta_ksi_est_err_tilt_1_4) -> [theta_ksi_est_err_tilt_1_4]
  Constant237/1 -> cal lumped observation error agent 4/2(w0)
  Mux132/1 -> ksi_d_est_2/3
  Demux70/3 -> Mux94/2
  Demux71/1 -> Mux95/1
  Mux133/1 -> ksi_d_est_3/1
  [eta_est_err_squ_2_node_3] -> cal theta_eta_est_err_tilt agent 3/3(eta_est_err_squ_2_node_3)
  cal abs 41/1(y) -> Mux115/1
  [ksi0] -> Add8/1
  cal lumped observation error agent 3/2(eta_est_err_tilt_3) -> [eta_est_err_tilt_3]
  [theta_ksi_est_err_tilt_2_vec] -> fixed-time distributed follower desire position observer agent 4/5(theta_ksi_est_err_tilt_2_vec)
  fixed-time distributed follower desire position observer agent 4/1(d_ksi_d_est_4) -> position observe Integrator 4/1
  Mux121/1 -> Interpreted MATLAB Function43/1
  Constant271/1 -> Mux124/3
  [theta_eta_est_err_tilt_1_vec] -> fixed-time distributed follower desire velocity observer agent 4/3(theta_eta_est_err_tilt_1_vec)
  [eta_d_est_vec] -> cal velocity estimate error/1(eta_d_est_vec)
  [ksi_est_err_tilt_vec] -> choose eta_est_err_tilt 11/1(x)
  Add2/1 -> Demux74/1
  Constant245/1 -> Mux115/2
  [theta_ksi_est_err_tilt_1_vec] -> fixed-time distributed follower desire position observer agent 5/4(theta_ksi_est_err_tilt_1_vec)
  Demux95/2 -> Mux134/2
  Constant241/1 -> Add6/2
  Demux97/1 -> Mux87/2
  [ksi_est_err_tilt_vec] -> cal theta_ksi_est_err_tilt agent 2/4(ksi_est_err_tilt_vec)
  [ksi_est_err_tilt_vec] -> choose eta_est_err_tilt 15/1(x)
  [eta0] -> Add1/1
  [eta0] -> Add4/1
  [ksi0] -> cal lumped observation error agent 4/4(ksi0)
  [theta_eta_est_err_tilt_2_vec] -> fixed-time distributed follower desire velocity observer agent 4/4(theta_eta_est_err_tilt_2_vec)
  Interpreted MATLAB Function41/1 -> trans to column41/1(x)
  Constant183/1 -> fixed-time distributed follower desire position observer agent 4/2(l2p)
  cal theta_eta_est_err_tilt agent 4/1(theta_eta_est_err_tilt_1_4) -> [theta_eta_est_err_tilt_1_4]
  Constant230/1 -> fixed-time distributed follower desire position observer agent 2/1(l1p)
  trans to column41/1(y) -> [eta_est_err_squ_2_node_1], Display76/1
  [eta_d_est_vec] -> fixed-time distributed follower desire position observer agent 2/3(eta_d_est_vec)
  Constant188/1 -> Add8/2
  fixed-time distributed follower desire velocity observer agent 1/1(d_eta_d_est_1) -> velocity observe Integrator 1/1
  [theta_ksi_est_err_tilt_2_vec] -> fixed-time distributed follower desire position observer agent 3/5(theta_ksi_est_err_tilt_2_vec)
  Mux125/1 -> Interpreted MATLAB Function48/1
  Demux96/1 -> Mux87/1
  [ksi_d_est_2] -> combine leader position estimaters/2(ksi_d_est_2)
  [ksi_d_est_vec] -> cal lumped observation error agent 1/3(ksi_d_est_vec)
  Demux97/2 -> Mux88/2
  [theta_eta_est_err_tilt_2_vec] -> fixed-time distributed follower desire velocity observer agent 1/4(theta_eta_est_err_tilt_2_vec)
  Demux83/2 -> ksi_est_err_3/2
  [ksi_est_err_tilt_3] -> "combine lumped follower observation error "/3(ksi_est_err_tilt_3)
  Constant198/1 -> cal theta_eta_est_err_tilt agent 5/1(alfa_theta)
  Demux71/3 -> Mux98/1
  Demux86/1 -> eta_est_err_1/1
  Constant283/1 -> cal theta_ksi_est_err_tilt agent 1/1(alfa_theta)
  [theta_eta_est_err_tilt_2_4] -> combine lumped follower velocity observation error/9(theta_eta_est_err_tilt_2_4)
  Mux101/1 -> eta_d_est_3/3
  Constant212/1 -> fixed-time distributed follower desire velocity observer agent 5/2(l2v)
  cal lumped observation error agent 2/2(eta_est_err_tilt_2) -> [eta_est_err_tilt_2]
  [theta_ksi_est_err_tilt_2_3] -> combine lumped follower position observation error/8(theta_ksi_est_err_tilt_2_3)
  [theta_eta_est_err_tilt_2_vec] -> fixed-time distributed follower desire velocity observer agent 3/4(theta_eta_est_err_tilt_2_vec)
  Constant194/1 -> cal theta_eta_est_err_tilt agent 2/1(alfa_theta)
  [ksi_est_err_squ_2_node_4] -> cal theta_ksi_est_err_tilt agent 4/3(ksi_est_err_squ_2_node_4)
  [eta_est_err_tilt_vec] -> choose eta_est_err_tilt 6/1(x)
  Interpreted MATLAB Function52/1 -> trans to column52/1(x)
  Demux87/3 -> eta_est_err_2/3
  Mux96/1 -> eta_d_est_2/2
  Demux79/3 -> Mux107/2
  cal lumped observation error agent 5/2(eta_est_err_tilt_5) -> [eta_est_err_tilt_5]
  cal abs 52/1(y) -> Mux109/1
  [ksi_est_err_squ_1_node_4] -> cal theta_ksi_est_err_tilt agent 4/2(ksi_est_err_squ_1_node_4)
  cal abs 54/1(y) -> Mux111/1
  [eta_est_err] -> divide eta_est_err/1(eta_est_err)
  velocity observe Integrator 1/1 -> [eta_d_est_1], Demux69/1
  [ksi_d_est_4] -> combine leader position estimaters/4(ksi_d_est_4)
  Demux76/2 -> Mux103/2
  Demux79/2 -> Mux106/2
  [theta_ksi_est_err_tilt_1_vec] -> fixed-time distributed follower desire position observer agent 4/4(theta_ksi_est_err_tilt_1_vec)
  [theta_ksi_est_err_tilt_2_2] -> combine lumped follower position observation error/7(theta_ksi_est_err_tilt_2_2)
  [eta0] -> cal lumped observation error agent 4/7(eta0)
  divide ksi_est_err/3(ksi_est_err_3) -> Demux83/1
  Demux95/1 -> Mux133/2
  divide eta_est_err/5(eta_est_err_5) -> Demux91/1
  Constant276/1 -> Mux127/3
  Demux96/3 -> Mux89/1
  [theta_eta_est_err_tilt_2_2] -> combine lumped follower velocity observation error/7(theta_eta_est_err_tilt_2_2)
  choose eta_est_err_tilt 2/1(y) -> cal abs 52/1(x)
  Constant196/1 -> cal theta_eta_est_err_tilt agent 4/1(alfa_theta)
  Demux92/1 -> Mux119/1
  Mux99/1 -> eta_d_est_3/1
  Constant284/1 -> cal theta_ksi_est_err_tilt agent 2/1(alfa_theta)
  Demux89/1 -> eta_est_err_3/1
  Interpreted MATLAB Function48/1 -> trans to column48/1(x)
  Constant257/1 -> Mux112/3
  Constant258/1 -> Mux116/2
  Demux83/1 -> ksi_est_err_3/1
  Demux81/3 -> ksi_est_err_1/3
  [ksi_est_err_squ_2_node_5] -> cal theta_ksi_est_err_tilt agent 5/3(ksi_est_err_squ_2_node_5)
  Interpreted MATLAB Function42/1 -> trans to column42/1(x)
  [theta_eta_est_err_tilt_1_vec] -> fixed-time distributed follower desire velocity observer agent 1/3(theta_eta_est_err_tilt_1_vec)
  Add9/1 -> Demux80/1
  [ksi_est_err_tilt_vec] -> cal theta_ksi_est_err_tilt agent 4/4(ksi_est_err_tilt_vec)
  Mux102/1 -> eta_d_est_4/1
  Constant208/1 -> Add5/2
  Demux68/1 -> Mux90/1
  cal abs 57/1(y) -> Mux112/1
  Constant195/1 -> cal theta_eta_est_err_tilt agent 3/1(alfa_theta)
  [eta_est_err_tilt_vec] -> cal theta_eta_est_err_tilt agent 5/4(eta_est_err_tilt_vec)
  Mux115/1 -> Interpreted MATLAB Function54/1
  [theta_ksi_est_err_tilt_1_vec] -> fixed-time distributed follower desire position observer agent 1/4(theta_ksi_est_err_tilt_1_vec)
  Demux80/2 -> Mux91/2
  Demux92/3 -> Mux132/1
  [eta_est_err_tilt_1] -> "combine lumped follower observation error "/6(eta_est_err_tilt_1)
  Constant182/1 -> fixed-time distributed follower desire position observer agent 1/2(l2p)
  Constant186/1 -> cal theta_ksi_est_err_tilt agent 5/1(alfa_theta)
  [ksi_est_err_tilt_vec] -> cal theta_ksi_est_err_tilt agent 5/4(ksi_est_err_tilt_vec)
  [eta_est_err_tilt_vec] -> choose eta_est_err_tilt 3/1(x)
  [ksi_est_err] -> divide ksi_est_err/1(ksi_est_err)
  trans to column53/1(y) -> [eta_est_err_squ_1_node_2], Display88/1
  Interpreted MATLAB Function43/1 -> trans to column43/1(x)
  Demux68/2 -> Mux91/1
  Constant269/1 -> Mux121/3
  Demux91/3 -> eta_est_err_5/3
  [ksi0] -> Add5/1
  Constant264/1 -> Mux118/3
  [ksi_d_est_1] -> combine leader position estimaters/1(ksi_d_est_1)
  [ksi_d_est_vec] -> cal lumped observation error agent 2/3(ksi_d_est_vec)
  cal theta_ksi_est_err_tilt agent 1/2(theta_ksi_est_err_tilt_2_1) -> [theta_ksi_est_err_tilt_2_1]
  Constant279/1 -> Mux129/2
  Demux94/1 -> Mux133/1
  cal abs 55/1(y) -> Mux110/1
  divide eta_est_err/3(eta_est_err_3) -> Demux89/1
  Interpreted MATLAB Function54/1 -> trans to column54/1(x)
  cal abs 46/1(y) -> Mux122/1
  Mux129/1 -> Interpreted MATLAB Function51/1
  Constant210/1 -> fixed-time distributed follower desire velocity observer agent 4/1(l1v)
  Mux126/1 -> Interpreted MATLAB Function45/1
  Demux89/3 -> eta_est_err_3/3
  choose eta_est_err_tilt 11/1(y) -> cal abs 43/1(x)
  divide ksi_est_err/5(ksi_est_err_5) -> Demux85/1
  [theta_eta_est_err_tilt_1_2] -> combine lumped follower velocity observation error/2(theta_eta_est_err_tilt_1_2)
  [eta_est_err_tilt_vec] -> choose eta_est_err_tilt 1/1(x)
  Demux79/1 -> Mux105/2
  choose eta_est_err_tilt 19/1(y) -> cal abs 51/1(x)
  [eta_d_est_vec] -> cal lumped observation error agent 3/6(eta_d_est_vec)
  Demux81/2 -> ksi_est_err_1/2
  trans to column42/1(y) -> [ksi_est_err_squ_2_node_1], Display77/1
  Interpreted MATLAB Function59/1 -> trans to column59/1(x)
  Demux84/3 -> ksi_est_err_4/3
  Mux122/1 -> Interpreted MATLAB Function44/1
  trans to column54/1(y) -> [eta_est_err_squ_1_node_1], Display93/1
  Demux70/1 -> Mux92/2
  [ksi_est_err_squ_2_node_2] -> cal theta_ksi_est_err_tilt agent 2/3(ksi_est_err_squ_2_node_2)
  [theta_eta_est_err_tilt_1_vec] -> fixed-time distributed follower desire velocity observer agent 3/3(theta_eta_est_err_tilt_1_vec)
  Demux91/2 -> eta_est_err_5/2
  [eta_est_err_squ_2_node_1] -> cal theta_eta_est_err_tilt agent 1/3(eta_est_err_squ_2_node_1)
  Demux90/3 -> eta_est_err_4/3
  [eta_d_est_vec] -> cal lumped observation error agent 4/6(eta_d_est_vec)
  Demux75/1 -> Mux102/1
  divide eta_est_err/1(eta_est_err_1) -> Demux86/1
  Mux106/1 -> eta_d_est_5/2
  Constant277/1 -> Mux125/2
  [eta_est_err_tilt_vec] -> choose eta_est_err_tilt 4/1(x)
  Constant193/1 -> cal theta_eta_est_err_tilt agent 1/1(alfa_theta)
  [ksi_est_err_tilt_vec] -> choose eta_est_err_tilt 20/1(x)
  Constant219/1 -> fixed-time distributed follower desire position observer agent 2/2(l2p)
  Constant184/1 -> cal theta_ksi_est_err_tilt agent 3/1(alfa_theta)
  Demux97/3 -> Mux89/2
  Constant253/1 -> Mux110/3
  [ksi_est_err_tilt_vec] -> choose eta_est_err_tilt 17/1(x)
  Mux116/1 -> Interpreted MATLAB Function58/1
  Constant185/1 -> cal theta_ksi_est_err_tilt agent 4/1(alfa_theta)
  Mux92/1 -> eta_d_est_1/1
  [theta_ksi_est_err_tilt_1_1] -> combine lumped follower position observation error/1(theta_ksi_est_err_tilt_1_1)
  [ksi_est_err] -> To Workspace17/1
  [ksi_d_est_vec] -> To Workspace18/1
  [eta_d_est_vec] -> To Workspace/1
  [eta_est_err] -> To Workspace22/1
  [ksi_d_est_vec] -> cal formation tracking position and velocity errors/2(ksi_d_est_vec)
  [ksi_i_vec] -> cal formation tracking position and velocity errors/1(ksi_i_vec)
  [eta_i_vec] -> cal formation tracking position and velocity errors/3(eta_i_vec)
  [eta_d_est_vec] -> cal formation tracking position and velocity errors/4(eta_d_est_vec)
  cal formation tracking position and velocity errors/1(err_ksi_vec) -> [err_ksi_vec]
  cal formation tracking position and velocity errors/2(err_eta_vec) -> [err_eta_vec]
  combine lumped follower velocity observation error/1(theta_eta_est_err_tilt_1_vec) -> [theta_eta_est_err_tilt_1_vec]
  combine lumped follower velocity observation error/2(theta_eta_est_err_tilt_2_vec) -> [theta_eta_est_err_tilt_2_vec]
  combine lumped follower position observation error/1(theta_ksi_est_err_tilt_1_vec) -> [theta_ksi_est_err_tilt_1_vec]
  combine lumped follower position observation error/2(theta_ksi_est_err_tilt_2_vec) -> [theta_ksi_est_err_tilt_2_vec]
  cal position estimate error/1(ksi_est_err) -> [ksi_est_err]
  combine leader position estimaters/1(ksi_d_est_vec) -> [ksi_d_est_vec]
  cal velocity estimate error/1(eta_est_err) -> [eta_est_err]
  combine follower desire velocity estimaters/1(eta_d_est_vec) -> [eta_d_est_vec]
  "combine lumped follower observation error "/1(ksi_est_err_tilt_vec) -> [ksi_est_err_tilt_vec]
  "combine lumped follower observation error "/2(eta_est_err_tilt_vec) -> [eta_est_err_tilt_vec]
  combine ui/1(ui) -> [ui]
  [d_chi_vec] -> cal ui agent 1/3(d_chi_vec)
  [sigma_v_vec] -> To Workspace19/1
  leader control input/1(u0) -> [u0]
  Constant/1 -> leader control input/2(T1)
  Clock/1 -> [tsim]
  Constant67/1 -> leader control input/6(Rx2)
  Constant68/1 -> leader control input/7(Ry2)
  Constant69/1 -> leader control input/8(Rz2)
  Constant64/1 -> leader control input/3(T2)
  Constant65/1 -> leader control input/4(R0)
  Constant66/1 -> leader control input/5(R1)
  [tsim] -> leader control input/1(t)
  Constant131/1 -> process velocity/1(T0)
  Demux1/1 -> ksi_0/1
  Constant73/1 -> process velocity/5(PZ1)
  Constant72/1 -> process velocity/4(PZ0)
  Step/1 -> leader eta0 Integrator/2
  leader eta0 Integrator/1 -> [eta0], leader ksi0 Integrator/1
  Constant134/1 -> process velocity/8(Rx2)
  Constant133/1 -> process velocity/9(Ry2)
  [eta0] -> Demux22/1
  Constant70/1 -> process velocity/3(T2)
  [ksi0] -> Demux1/1
  [tsim] -> process velocity/11(t)
  Demux22/2 -> eta_0/2
  Demux1/2 -> ksi_0/2
  Demux22/3 -> eta_0/3
  Constant130/1 -> process velocity/7(R1)
  Demux22/1 -> eta_0/1
  Constant129/1 -> process velocity/6(R0)
  Constant132/1 -> process velocity/10(Rz2)
  process velocity/1(V_init_out) -> [V_init_out]
  [V_init_out] -> leader eta0 Integrator/3
  Demux1/3 -> ksi_0/3
  leader ksi0 Integrator/1 -> [ksi0]
  Constant71/1 -> process velocity/2(T1)
  [u0] -> leader eta0 Integrator/1
  Constant225/1 -> set desire formation configuration/10(theta0)
  Constant231/1 -> set desire formation configuration/11(kai_1_t)
  [tsim] -> set desire formation configuration/15(t)
  Constant222/1 -> set desire formation configuration/8(Z2)
  Constant238/1 -> set desire formation configuration/13(T1)
  Constant234/1 -> set desire formation configuration/3(X3)
  Constant226/1 -> set desire formation configuration/9(Z3)
  Constant138/1 -> set desire formation configuration/5(Y2)
  Constant136/1 -> set desire formation configuration/2(X2)
  Constant135/1 -> set desire formation configuration/1(X1)
  set desire formation configuration/1(delta_ksi_vec) -> [delta_ksi_vec]
  Constant239/1 -> set desire formation configuration/14(T12)
  Constant221/1 -> set desire formation configuration/7(Z1)
  Constant229/1 -> set desire formation configuration/6(Y3)
  set desire formation configuration/2(delta_eta_vec) -> [delta_eta_vec]
  Constant235/1 -> set desire formation configuration/12(kai_3_t)
  Constant137/1 -> set desire formation configuration/4(Y1)
  desire formation position and velocity/1(pos_i_des) -> [pos_i_des]
  [delta_eta_vec] -> desire formation position and velocity/4(delta_eta_vec)
  [eta0] -> desire formation position and velocity/2(eta0)
  [delta_ksi_vec] -> desire formation position and velocity/3(delta_ksi_vec)
  [ksi0] -> desire formation position and velocity/1(ksi0)
  desire formation position and velocity/2(vel_i_des) -> [vel_i_des]
  [delta_eta_vec] -> cal lumped observation error agent 1/8(delta_eta_vec)
  [delta_ksi_vec] -> cal lumped observation error agent 1/5(delta_ksi_vec)
  [delta_ksi_vec] -> cal lumped observation error agent 3/5(delta_ksi_vec)
  [delta_eta_vec] -> cal lumped observation error agent 3/8(delta_eta_vec)
  [delta_ksi_vec] -> cal lumped observation error agent 5/5(delta_ksi_vec)
  [delta_eta_vec] -> cal lumped observation error agent 5/8(delta_eta_vec)
  [delta_ksi_vec] -> cal lumped observation error agent 2/5(delta_ksi_vec)
  [delta_eta_vec] -> cal lumped observation error agent 2/8(delta_eta_vec)
  [delta_ksi_vec] -> cal lumped observation error agent 4/5(delta_ksi_vec)
  [delta_eta_vec] -> cal lumped observation error agent 4/8(delta_eta_vec)
  [delta_ksi_vec] -> follower tracking error agent 1/1(delta_ksi_vec)
  [delta_eta_vec] -> follower tracking error agent 1/2(delta_eta_vec)
  [delta_eta_vec] -> follower tracking error agent 2/2(delta_eta_vec)
  [delta_ksi_vec] -> follower tracking error agent 2/1(delta_ksi_vec)
  [delta_ksi_vec] -> follower tracking error agent 4/1(delta_ksi_vec)
  [delta_eta_vec] -> follower tracking error agent 4/2(delta_eta_vec)
  [delta_ksi_vec] -> follower tracking error agent 3/1(delta_ksi_vec)
  [delta_eta_vec] -> follower tracking error agent 3/2(delta_eta_vec)
  [delta_ksi_vec] -> follower tracking error agent 5/1(delta_ksi_vec)
  [delta_eta_vec] -> follower tracking error agent 5/2(delta_eta_vec)
  [delta_ksi_vec] -> To Workspace20/1
  [delta_eta_vec] -> To Workspace21/1
  [delta_eta_vec] -> cal velocity estimate error/3(delta_eta_vec)
  [delta_ksi_vec] -> cal position estimate error/3(delta_ksi_vec)
  Constant243/1 -> generate translational disturbance agent 1/3(dp_phi_t)
  Constant244/1 -> generate translational disturbance agent 1/2(dp_ff_t)
  Constant285/1 -> generate translational disturbance agent 1/1(dp_aa_t)
  Constant288/1 -> generate translational disturbance agent 2/1(dp_aa_t)
  Constant287/1 -> generate translational disturbance agent 2/2(dp_ff_t)
  [tsim] -> generate translational disturbance agent 2/4(t)
  generate translational disturbance agent 2/1(dp_2) -> [dp_2]
  Constant286/1 -> generate translational disturbance agent 2/3(dp_phi_t)
  Constant289/1 -> generate translational disturbance agent 3/3(dp_phi_t)
  Constant290/1 -> generate translational disturbance agent 3/2(dp_ff_t)
  generate translational disturbance agent 3/1(dp_3) -> [dp_3]
  [tsim] -> generate translational disturbance agent 3/4(t)
  Constant291/1 -> generate translational disturbance agent 3/1(dp_aa_t)
  [tsim] -> generate translational disturbance agent 4/4(t)
  generate translational disturbance agent 4/1(dp_4) -> [dp_4]
  Constant294/1 -> generate translational disturbance agent 4/1(dp_aa_t)
  Constant293/1 -> generate translational disturbance agent 4/2(dp_ff_t)
  Constant292/1 -> generate translational disturbance agent 4/3(dp_phi_t)
  Constant297/1 -> generate translational disturbance agent 5/1(dp_aa_t)
  Constant295/1 -> generate translational disturbance agent 5/3(dp_phi_t)
  [tsim] -> generate translational disturbance agent 5/4(t)
  Constant296/1 -> generate translational disturbance agent 5/2(dp_ff_t)
  generate translational disturbance agent 5/1(dp_5) -> [dp_5]
